simulink model "c00006M_harness"  (R2018a)
settings: Solver=FixedStepAuto  StartTime=0.0  StopTime=300  FixedStep=0.1  RelTol=1e-3
undefined symbols (not defined in the file): A1, hmax, PriorityTank, R1, R2, sigbuilder_block, TempThreshold
(part 1 of 66)
settings Model: Creator=aarrieta  LastModifiedBy=umarkiegi

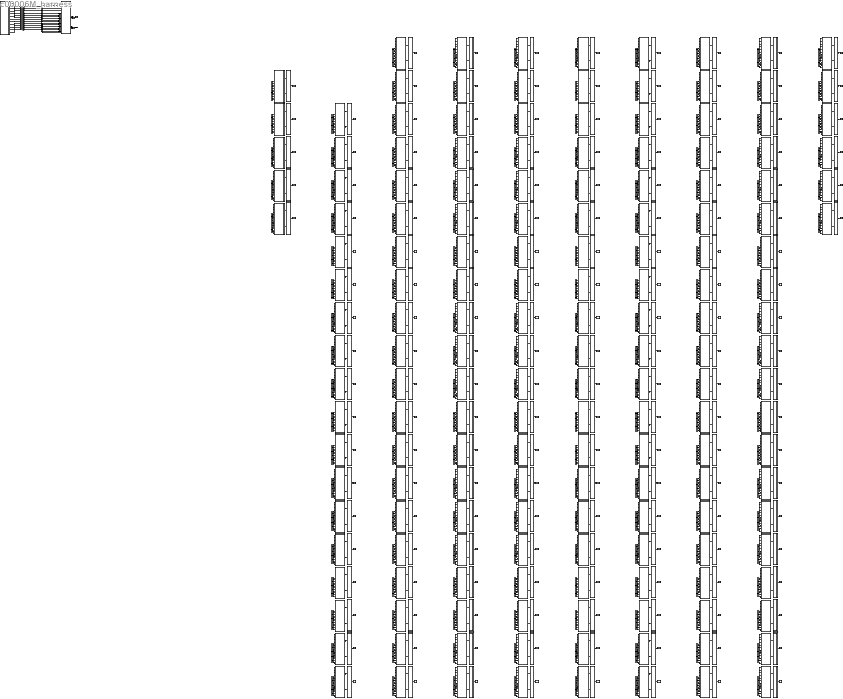
== system c00006M_harness ==
  CPSUT : Subsystem
  Eval100 : Subsystem
  Eval101 : Subsystem
  Eval102 : Subsystem
  Eval103 : Subsystem
  Eval104 : Subsystem
  Eval105 : Subsystem
  Eval106 : Subsystem
  Eval107 : Subsystem
  Eval108 : Subsystem
  Eval109 : Subsystem
  Eval110 : Subsystem
  Eval111 : Subsystem
  Eval112 : Subsystem
  Eval113 : Subsystem
  Eval114 : Subsystem
  Eval115 : Subsystem
  Eval116 : Subsystem
  Eval117 : Subsystem
  Eval118 : Subsystem
  Eval119 : Subsystem
  Eval120 : Subsystem
  Eval121 : Subsystem
  Eval122 : Subsystem
  Eval123 : Subsystem
  Eval124 : Subsystem
  Eval125 : Subsystem
  Eval126 : Subsystem
  Eval127 : Subsystem
  Eval128 : Subsystem
  Eval129 : Subsystem
  Eval130 : Subsystem
  Eval131 : Subsystem
  Eval132 : Subsystem
  Eval133 : Subsystem
  Eval134 : Subsystem
  Eval135 : Subsystem
  Eval136 : Subsystem
  Eval137 : Subsystem
  Eval138 : Subsystem
  Eval139 : Subsystem
  Eval140 : Subsystem
  Eval141 : Subsystem
  Eval142 : Subsystem
  Eval143 : Subsystem
  Eval144 : Subsystem
  Eval145 : Subsystem
  Eval146 : Subsystem
  Eval147 : Subsystem
  Eval148 : Subsystem
  Eval149 : Subsystem
  Eval150 : Subsystem
  Eval151 : Subsystem
  Eval152 : Subsystem
  Eval153 : Subsystem
  Eval154 : Subsystem
  Eval155 : Subsystem
  Eval156 : Subsystem
  Eval157 : Subsystem
  Eval158 : Subsystem
  Eval159 : Subsystem
  Eval160 : Subsystem
  Eval161 : Subsystem
  Eval162 : Subsystem
  Eval163 : Subsystem
  Eval164 : Subsystem
  Eval165 : Subsystem
  Eval166 : Subsystem
  Eval167 : Subsystem
  Eval168 : Subsystem
  Eval169 : Subsystem
  Eval170 : Subsystem
  Eval171 : Subsystem
  Eval172 : Subsystem
  Eval173 : Subsystem
  Eval174 : Subsystem
  Eval175 : Subsystem
  Eval176 : Subsystem
  Eval177 : Subsystem
  Eval178 : Subsystem
  Eval179 : Subsystem
  Eval180 : Subsystem
  Eval181 : Subsystem
  Eval182 : Subsystem
  Eval183 : Subsystem
  Eval184 : Subsystem
  Eval185 : Subsystem
  Eval186 : Subsystem
  Eval187 : Subsystem
  Eval188 : Subsystem
  Eval189 : Subsystem
  Eval190 : Subsystem
  Eval191 : Subsystem
  Eval192 : Subsystem
  Eval193 : Subsystem
  Eval194 : Subsystem
  Eval195 : Subsystem
  Eval196 : Subsystem
  Eval197 : Subsystem
  Eval198 : Subsystem
  Eval199 : Subsystem
  Eval200 : Subsystem
  Eval201 : Subsystem
  Eval202 : Subsystem
  Eval203 : Subsystem
  Eval204 : Subsystem
  Eval205 : Subsystem
  Eval206 : Subsystem
  Eval207 : Subsystem
  Eval208 : Subsystem
  Eval209 : Subsystem
  Eval210 : Subsystem
  Eval211 : Subsystem
  Eval212 : Subsystem
  Eval213 : Subsystem
  Eval214 : Subsystem
  Eval215 : Subsystem
  Eval216 : Subsystem
  Eval217 : Subsystem
  Eval218 : Subsystem
  Eval219 : Subsystem
  Eval220 : Subsystem
  Eval221 : Subsystem
  Eval222 : Subsystem
  Eval223 : Subsystem
  Eval224 : Subsystem
  Eval225 : Subsystem
  Eval226 : Subsystem
  Eval227 : Subsystem
  Eval228 : Subsystem
  Eval229 : Subsystem
  Eval230 : Subsystem
  Eval231 : Subsystem
  Eval232 : Subsystem
  Eval233 : Subsystem
  Eval234 : Subsystem
  Eval235 : Subsystem
  Eval236 : Subsystem
  Eval237 : Subsystem
  Eval238 : Subsystem
  Eval239 : Subsystem
  Eval240 : Subsystem
  Eval241 : Subsystem
  Eval242 : Subsystem
  Eval243 : Subsystem
  Eval244 : Subsystem
  Eval245 : Subsystem
  Eval61 : Subsystem
  Eval62 : Subsystem
  Eval63 : Subsystem
  Eval64 : Subsystem
  Eval65 : Subsystem
  Eval82 : Subsystem
  Eval83 : Subsystem
  Eval84 : Subsystem
  Eval85 : Subsystem
  Eval86 : Subsystem
  Eval87 : Subsystem
  Eval88 : Subsystem
  Eval89 : Subsystem
  Eval90 : Subsystem
  Eval91 : Subsystem
  Eval92 : Subsystem
  Eval93 : Subsystem
  Eval94 : Subsystem
  Eval95 : Subsystem
  Eval96 : Subsystem
  Eval97 : Subsystem
  Eval98 : Subsystem
  Eval99 : Subsystem
  Inputs : Subsystem  Tag=STV Subsys  LoadFcn=sigbuilder_block('load');  StartFcn=sigbuilder_block('start');  StopFcn=sigbuilder_block('stop');  ClipboardFcn=sigbuilder_block('clipboard');  mask(Sigbuilder block){tuvar=[0:10]}
      mask init:
      | if ~strcmp(get_param(bdroot(gcb),'SimulationStatus'),'stopped'),tuvar = sigbuilder_block('maskInit'); end
      settings: CopyFcn=sigbuilder_block('copy');  DeleteFcn=sigbuilder_block('delete');  ModelCloseFcn=sigbuilder_block('modelClose');  PreSaveFcn=sigbuilder_block('preSave');  PauseFcn=sigbuilder_block('pause');  ContinueFcn=sigbuilder_block('continue');  NameChangeFcn=sigbuilder_block('namechange');  OpenFcn=sigbuilder_block('open',[276.75 163.5 675.75 486.75 ]);  CloseFcn=sigbuilder_block('close');
      mask Display: plot(0, 0, 100, 100,[2, 2, 32, 32, 2], [68, 8, 8, 68, 68],[32, 2], [38, 38], [32, 19, 2],[53, 60, 44], [32, 17, 17, 2],[16, 16, 31, 31]);txt = getActiveGroup(gcbh);text(2, 100, txt,'verticalAlignment', 'top');
  M062 : Subsystem
  M063 : Subsystem
  M064 : Subsystem
  M065 : Subsystem
  M066 : Subsystem
  M083 : Subsystem
  M084 : Subsystem
  M085 : Subsystem
  M086 : Subsystem
  M087 : Subsystem
  M088 : Subsystem
  M089 : Subsystem
  M090 : Subsystem
  M091 : Subsystem
  M092 : Subsystem
  M093 : Subsystem
  M094 : Subsystem
  M095 : Subsystem
  M096 : Subsystem
  M097 : Subsystem
  M098 : Subsystem
  M099 : Subsystem
  M100 : Subsystem
  M101 : Subsystem
  M102 : Subsystem
  M103 : Subsystem
  M104 : Subsystem
  M105 : Subsystem
  M106 : Subsystem
  M107 : Subsystem
  M108 : Subsystem
  M109 : Subsystem
  M110 : Subsystem
  M111 : Subsystem
  M112 : Subsystem
  M113 : Subsystem
  M114 : Subsystem
  M115 : Subsystem
  M116 : Subsystem
  M117 : Subsystem
  M118 : Subsystem
  M119 : Subsystem
  M120 : Subsystem
  M121 : Subsystem
  M122 : Subsystem
  M123 : Subsystem
  M124 : Subsystem
  M125 : Subsystem
  M126 : Subsystem
  M127 : Subsystem
  M128 : Subsystem
  M129 : Subsystem
  M130 : Subsystem
  M131 : Subsystem
  M132 : Subsystem
  M133 : Subsystem
  M134 : Subsystem
  M135 : Subsystem
  M136 : Subsystem
  M137 : Subsystem
  M138 : Subsystem
  M139 : Subsystem
  M140 : Subsystem
  M141 : Subsystem
  M142 : Subsystem
  M143 : Subsystem
  M144 : Subsystem
  M145 : Subsystem
  M146 : Subsystem
  M147 : Subsystem
  M148 : Subsystem
  M149 : Subsystem
  M150 : Subsystem
  M151 : Subsystem
  M152 : Subsystem
  M153 : Subsystem
  M154 : Subsystem
  M155 : Subsystem
  M156 : Subsystem
  M157 : Subsystem
  M158 : Subsystem
  M159 : Subsystem
  M160 : Subsystem
  M161 : Subsystem
  M162 : Subsystem
  M163 : Subsystem
  M164 : Subsystem
  M165 : Subsystem
  M166 : Subsystem
  M167 : Subsystem
  M168 : Subsystem
  M169 : Subsystem
  M170 : Subsystem
  M171 : Subsystem
  M172 : Subsystem
  M173 : Subsystem
  M174 : Subsystem
  M175 : Subsystem
  M176 : Subsystem
  M177 : Subsystem
  M178 : Subsystem
  M179 : Subsystem
  M180 : Subsystem
  M181 : Subsystem
  M182 : Subsystem
  M183 : Subsystem
  M184 : Subsystem
  M185 : Subsystem
  M186 : Subsystem
  M187 : Subsystem
  M188 : Subsystem
  M189 : Subsystem
  M190 : Subsystem
  M191 : Subsystem
  M192 : Subsystem
  M193 : Subsystem
  M194 : Subsystem
  M195 : Subsystem
  M196 : Subsystem
  M197 : Subsystem
  M198 : Subsystem
  M199 : Subsystem
  M200 : Subsystem
  M201 : Subsystem
  M202 : Subsystem
  M203 : Subsystem
  M204 : Subsystem
  M205 : Subsystem
  M206 : Subsystem
  M207 : Subsystem
  M208 : Subsystem
  M209 : Subsystem
  M210 : Subsystem
  M211 : Subsystem
  M212 : Subsystem
  M213 : Subsystem
  M214 : Subsystem
  M215 : Subsystem
  M216 : Subsystem
  M217 : Subsystem
  M218 : Subsystem
  M219 : Subsystem
  M220 : Subsystem
  M221 : Subsystem
  M222 : Subsystem
  M223 : Subsystem
  M224 : Subsystem
  M225 : Subsystem
  M226 : Subsystem
  M227 : Subsystem
  M228 : Subsystem
  M229 : Subsystem
  M230 : Subsystem
  M231 : Subsystem
  M232 : Subsystem
  M233 : Subsystem
  M234 : Subsystem
  M235 : Subsystem
  M236 : Subsystem
  M237 : Subsystem
  M238 : Subsystem
  M239 : Subsystem
  M240 : Subsystem
  M241 : Subsystem
  M242 : Subsystem
  M243 : Subsystem
  M244 : Subsystem
  M245 : Subsystem
  M246 : Subsystem
  To Workspace100 : ToWorkspace  VariableName=mutant101  SampleTime=-1
  To Workspace101 : ToWorkspace  VariableName=mutant102  SampleTime=-1
  To Workspace102 : ToWorkspace  VariableName=mutant103  SampleTime=-1
  To Workspace103 : ToWorkspace  VariableName=mutant104  SampleTime=-1
  To Workspace104 : ToWorkspace  VariableName=mutant105  SampleTime=-1
  To Workspace105 : ToWorkspace  VariableName=mutant106  SampleTime=-1
  To Workspace106 : ToWorkspace  VariableName=mutant107  SampleTime=-1
  To Workspace107 : ToWorkspace  VariableName=mutant108  SampleTime=-1
  To Workspace108 : ToWorkspace  VariableName=mutant109  SampleTime=-1
  To Workspace109 : ToWorkspace  VariableName=mutant110  SampleTime=-1
  To Workspace110 : ToWorkspace  VariableName=mutant111  SampleTime=-1
  To Workspace111 : ToWorkspace  VariableName=mutant112  SampleTime=-1
  To Workspace112 : ToWorkspace  VariableName=mutant113  SampleTime=-1
  To Workspace113 : ToWorkspace  VariableName=mutant114  SampleTime=-1
  To Workspace114 : ToWorkspace  VariableName=mutant115  SampleTime=-1
  To Workspace115 : ToWorkspace  VariableName=mutant116  SampleTime=-1
  To Workspace116 : ToWorkspace  VariableName=mutant117  SampleTime=-1
  To Workspace117 : ToWorkspace  VariableName=mutant118  SampleTime=-1
  To Workspace118 : ToWorkspace  VariableName=mutant119  SampleTime=-1
  To Workspace119 : ToWorkspace  VariableName=mutant120  SampleTime=-1
  To Workspace120 : ToWorkspace  VariableName=mutant121  SampleTime=-1
  To Workspace121 : ToWorkspace  VariableName=mutant122  SampleTime=-1
  To Workspace122 : ToWorkspace  VariableName=mutant123  SampleTime=-1
  To Workspace123 : ToWorkspace  VariableName=mutant124  SampleTime=-1
  To Workspace124 : ToWorkspace  VariableName=mutant125  SampleTime=-1
  To Workspace125 : ToWorkspace  VariableName=mutant126  SampleTime=-1
  To Workspace126 : ToWorkspace  VariableName=mutant127  SampleTime=-1
  To Workspace127 : ToWorkspace  VariableName=mutant128  SampleTime=-1
  To Workspace128 : ToWorkspace  VariableName=mutant129  SampleTime=-1
  To Workspace129 : ToWorkspace  VariableName=mutant130  SampleTime=-1
  To Workspace130 : ToWorkspace  VariableName=mutant131  SampleTime=-1
  To Workspace131 : ToWorkspace  VariableName=mutant132  SampleTime=-1
  To Workspace132 : ToWorkspace  VariableName=mutant133  SampleTime=-1
  To Workspace133 : ToWorkspace  VariableName=mutant134  SampleTime=-1
  To Workspace134 : ToWorkspace  VariableName=mutant135  SampleTime=-1
  To Workspace135 : ToWorkspace  VariableName=mutant136  SampleTime=-1
  To Workspace136 : ToWorkspace  VariableName=mutant137  SampleTime=-1
  To Workspace137 : ToWorkspace  VariableName=mutant138  SampleTime=-1
  To Workspace138 : ToWorkspace  VariableName=mutant139  SampleTime=-1
  To Workspace139 : ToWorkspace  VariableName=mutant140  SampleTime=-1
  To Workspace140 : ToWorkspace  VariableName=mutant141  SampleTime=-1
  To Workspace141 : ToWorkspace  VariableName=mutant142  SampleTime=-1
  To Workspace142 : ToWorkspace  VariableName=mutant143  SampleTime=-1
  To Workspace143 : ToWorkspace  VariableName=mutant144  SampleTime=-1
  To Workspace144 : ToWorkspace  VariableName=mutant145  SampleTime=-1
  To Workspace145 : ToWorkspace  VariableName=mutant146  SampleTime=-1
  To Workspace146 : ToWorkspace  VariableName=mutant147  SampleTime=-1
  To Workspace147 : ToWorkspace  VariableName=mutant148  SampleTime=-1
  To Workspace148 : ToWorkspace  VariableName=mutant149  SampleTime=-1
  To Workspace149 : ToWorkspace  VariableName=mutant150  SampleTime=-1
  To Workspace150 : ToWorkspace  VariableName=mutant151  SampleTime=-1
  To Workspace151 : ToWorkspace  VariableName=mutant152  SampleTime=-1
  To Workspace152 : ToWorkspace  VariableName=mutant153  SampleTime=-1
  To Workspace153 : ToWorkspace  VariableName=mutant154  SampleTime=-1
  To Workspace154 : ToWorkspace  VariableName=mutant155  SampleTime=-1
  To Workspace155 : ToWorkspace  VariableName=mutant156  SampleTime=-1
  To Workspace156 : ToWorkspace  VariableName=mutant157  SampleTime=-1
  To Workspace157 : ToWorkspace  VariableName=mutant158  SampleTime=-1
  To Workspace158 : ToWorkspace  VariableName=mutant159  SampleTime=-1
  To Workspace159 : ToWorkspace  VariableName=mutant160  SampleTime=-1
  To Workspace160 : ToWorkspace  VariableName=mutant161  SampleTime=-1
  To Workspace161 : ToWorkspace  VariableName=mutant162  SampleTime=-1
  To Workspace162 : ToWorkspace  VariableName=mutant163  SampleTime=-1
  To Workspace163 : ToWorkspace  VariableName=mutant164  SampleTime=-1
  To Workspace164 : ToWorkspace  VariableName=mutant165  SampleTime=-1
  To Workspace165 : ToWorkspace  VariableName=mutant166  SampleTime=-1
  To Workspace166 : ToWorkspace  VariableName=mutant167  SampleTime=-1
  To Workspace167 : ToWorkspace  VariableName=mutant168  SampleTime=-1
  To Workspace168 : ToWorkspace  VariableName=mutant169  SampleTime=-1
  To Workspace169 : ToWorkspace  VariableName=mutant170  SampleTime=-1
  To Workspace170 : ToWorkspace  VariableName=mutant171  SampleTime=-1
  To Workspace171 : ToWorkspace  VariableName=mutant172  SampleTime=-1
  To Workspace172 : ToWorkspace  VariableName=mutant173  SampleTime=-1
  To Workspace173 : ToWorkspace  VariableName=mutant174  SampleTime=-1
  To Workspace174 : ToWorkspace  VariableName=mutant175  SampleTime=-1
  To Workspace175 : ToWorkspace  VariableName=mutant176  SampleTime=-1
  To Workspace176 : ToWorkspace  VariableName=mutant177  SampleTime=-1
  To Workspace177 : ToWorkspace  VariableName=mutant178  SampleTime=-1
  To Workspace178 : ToWorkspace  VariableName=mutant179  SampleTime=-1
  To Workspace179 : ToWorkspace  VariableName=mutant180  SampleTime=-1
  To Workspace180 : ToWorkspace  VariableName=mutant181  SampleTime=-1
  To Workspace181 : ToWorkspace  VariableName=mutant182  SampleTime=-1
  To Workspace182 : ToWorkspace  VariableName=mutant183  SampleTime=-1
  To Workspace183 : ToWorkspace  VariableName=mutant184  SampleTime=-1
  To Workspace184 : ToWorkspace  VariableName=mutant185  SampleTime=-1
  To Workspace185 : ToWorkspace  VariableName=mutant186  SampleTime=-1
  To Workspace186 : ToWorkspace  VariableName=mutant187  SampleTime=-1
  To Workspace187 : ToWorkspace  VariableName=mutant188  SampleTime=-1
  To Workspace188 : ToWorkspace  VariableName=mutant189  SampleTime=-1
  To Workspace189 : ToWorkspace  VariableName=mutant190  SampleTime=-1
  To Workspace190 : ToWorkspace  VariableName=mutant191  SampleTime=-1
  To Workspace191 : ToWorkspace  VariableName=mutant192  SampleTime=-1
  To Workspace192 : ToWorkspace  VariableName=mutant193  SampleTime=-1
  To Workspace193 : ToWorkspace  VariableName=mutant194  SampleTime=-1
  To Workspace194 : ToWorkspace  VariableName=mutant195  SampleTime=-1
  To Workspace195 : ToWorkspace  VariableName=mutant196  SampleTime=-1
  To Workspace196 : ToWorkspace  VariableName=mutant197  SampleTime=-1
  To Workspace197 : ToWorkspace  VariableName=mutant198  SampleTime=-1
  To Workspace198 : ToWorkspace  VariableName=mutant199  SampleTime=-1
  To Workspace199 : ToWorkspace  VariableName=mutant200  SampleTime=-1
  To Workspace200 : ToWorkspace  VariableName=mutant201  SampleTime=-1
  To Workspace201 : ToWorkspace  VariableName=mutant202  SampleTime=-1
  To Workspace202 : ToWorkspace  VariableName=mutant203  SampleTime=-1
  To Workspace203 : ToWorkspace  VariableName=mutant204  SampleTime=-1
  To Workspace204 : ToWorkspace  VariableName=mutant205  SampleTime=-1
  To Workspace205 : ToWorkspace  VariableName=mutant206  SampleTime=-1
  To Workspace206 : ToWorkspace  VariableName=mutant207  SampleTime=-1
  To Workspace207 : ToWorkspace  VariableName=mutant208  SampleTime=-1
  To Workspace208 : ToWorkspace  VariableName=mutant209  SampleTime=-1
  To Workspace209 : ToWorkspace  VariableName=mutant210  SampleTime=-1
  To Workspace210 : ToWorkspace  VariableName=mutant211  SampleTime=-1
  To Workspace211 : ToWorkspace  VariableName=mutant212  SampleTime=-1
  To Workspace212 : ToWorkspace  VariableName=mutant213  SampleTime=-1
  To Workspace213 : ToWorkspace  VariableName=mutant214  SampleTime=-1
  To Workspace214 : ToWorkspace  VariableName=mutant215  SampleTime=-1
  To Workspace215 : ToWorkspace  VariableName=mutant216  SampleTime=-1
  To Workspace216 : ToWorkspace  VariableName=mutant217  SampleTime=-1
  To Workspace217 : ToWorkspace  VariableName=mutant218  SampleTime=-1
  To Workspace218 : ToWorkspace  VariableName=mutant219  SampleTime=-1
  To Workspace219 : ToWorkspace  VariableName=mutant220  SampleTime=-1
  To Workspace220 : ToWorkspace  VariableName=mutant221  SampleTime=-1
  To Workspace221 : ToWorkspace  VariableName=mutant222  SampleTime=-1
  To Workspace222 : ToWorkspace  VariableName=mutant223  SampleTime=-1
  To Workspace223 : ToWorkspace  VariableName=mutant224  SampleTime=-1
  To Workspace224 : ToWorkspace  VariableName=mutant225  SampleTime=-1
  To Workspace225 : ToWorkspace  VariableName=mutant226  SampleTime=-1
  To Workspace226 : ToWorkspace  VariableName=mutant227  SampleTime=-1
  To Workspace227 : ToWorkspace  VariableName=mutant228  SampleTime=-1
  To Workspace228 : ToWorkspace  VariableName=mutant229  SampleTime=-1
  To Workspace229 : ToWorkspace  VariableName=mutant230  SampleTime=-1
  To Workspace230 : ToWorkspace  VariableName=mutant231  SampleTime=-1
  To Workspace231 : ToWorkspace  VariableName=mutant232  SampleTime=-1
  To Workspace232 : ToWorkspace  VariableName=mutant233  SampleTime=-1
  To Workspace233 : ToWorkspace  VariableName=mutant234  SampleTime=-1
  To Workspace234 : ToWorkspace  VariableName=mutant235  SampleTime=-1
  To Workspace235 : ToWorkspace  VariableName=mutant236  SampleTime=-1
  To Workspace236 : ToWorkspace  VariableName=mutant237  SampleTime=-1
  To Workspace237 : ToWorkspace  VariableName=mutant238  SampleTime=-1
  To Workspace238 : ToWorkspace  VariableName=mutant239  SampleTime=-1
  To Workspace239 : ToWorkspace  VariableName=mutant240  SampleTime=-1
  To Workspace240 : ToWorkspace  VariableName=mutant241  SampleTime=-1
  To Workspace241 : ToWorkspace  VariableName=mutant242  SampleTime=-1
  To Workspace242 : ToWorkspace  VariableName=mutant243  SampleTime=-1
  To Workspace243 : ToWorkspace  VariableName=mutant244  SampleTime=-1
  To Workspace244 : ToWorkspace  VariableName=mutant245  SampleTime=-1
  To Workspace245 : ToWorkspace  VariableName=mutant246  SampleTime=-1
  To Workspace61 : ToWorkspace  VariableName=mutant062  SampleTime=-1
  To Workspace62 : ToWorkspace  VariableName=mutant063  SampleTime=-1
  To Workspace63 : ToWorkspace  VariableName=mutant064  SampleTime=-1
  To Workspace64 : ToWorkspace  VariableName=mutant065  SampleTime=-1
  To Workspace65 : ToWorkspace  VariableName=mutant066  SampleTime=-1
  To Workspace82 : ToWorkspace  VariableName=mutant083  SampleTime=-1
  To Workspace83 : ToWorkspace  VariableName=mutant084  SampleTime=-1
  To Workspace84 : ToWorkspace  VariableName=mutant085  SampleTime=-1
  To Workspace85 : ToWorkspace  VariableName=mutant086  SampleTime=-1
  To Workspace86 : ToWorkspace  VariableName=mutant087  SampleTime=-1
  To Workspace87 : ToWorkspace  VariableName=mutant088  SampleTime=-1
  To Workspace88 : ToWorkspace  VariableName=mutant089  SampleTime=-1
  To Workspace89 : ToWorkspace  VariableName=mutant090  SampleTime=-1
  To Workspace90 : ToWorkspace  VariableName=mutant091  SampleTime=-1
  To Workspace91 : ToWorkspace  VariableName=mutant092  SampleTime=-1
  To Workspace92 : ToWorkspace  VariableName=mutant093  SampleTime=-1
  To Workspace93 : ToWorkspace  VariableName=mutant094  SampleTime=-1
  To Workspace94 : ToWorkspace  VariableName=mutant095  SampleTime=-1
  To Workspace95 : ToWorkspace  VariableName=mutant096  SampleTime=-1
  To Workspace96 : ToWorkspace  VariableName=mutant097  SampleTime=-1
  To Workspace97 : ToWorkspace  VariableName=mutant098  SampleTime=-1
  To Workspace98 : ToWorkspace  VariableName=mutant099  SampleTime=-1
  To Workspace99 : ToWorkspace  VariableName=mutant100  SampleTime=-1
  dtc_CT2 : DataTypeConversion
  dtc_CT3 : DataTypeConversion
  dtc_E2 : DataTypeConversion
  dtc_E3 : DataTypeConversion
  dtc_EB2 : DataTypeConversion
  dtc_EB3 : DataTypeConversion
  dtc_F2 : DataTypeConversion
  dtc_F3 : DataTypeConversion
  dtc_MR2 : DataTypeConversion
  dtc_MR3 : DataTypeConversion
  dtc_T2 : DataTypeConversion
  dtc_T3 : DataTypeConversion
  LL2 : Outport
  LL3 : Outport  Port=2
  tag scope: out2=global, out3=global
  wires:
  CPSUT/1(LL2) -> [out2], LL2/1
  CPSUT/2(LL3) -> [out3], LL3/1
  [in7] -> M062/1(CT2)
  [in8] -> M062/2(F2)
  [in9] -> M062/3(E2)
  [in10] -> M062/4(MR2)
  [in11] -> M062/5(T2)
  [in12] -> M062/6(EB2)
  [in13] -> M062/7(CT3)
  [in14] -> M062/8(F3)
  [in15] -> M062/9(E3)
  [in16] -> M062/10(MR3)
  [in17] -> M062/11(T3)
  [in18] -> M062/12(EB3)
  M062/1(LL2) -> Eval61/1(In2)
  M062/2(LL3) -> Eval61/2(In3)
  Eval61/1(Out1) -> To Workspace61/1
  [in7] -> M063/1(CT2)
  [in8] -> M063/2(F2)
  [in9] -> M063/3(E2)
  [in10] -> M063/4(MR2)
  [in11] -> M063/5(T2)
  [in12] -> M063/6(EB2)
  [in13] -> M063/7(CT3)
  [in14] -> M063/8(F3)
  [in15] -> M063/9(E3)
  [in16] -> M063/10(MR3)
  [in17] -> M063/11(T3)
  [in18] -> M063/12(EB3)
  M063/1(LL2) -> Eval62/1(In2)
  M063/2(LL3) -> Eval62/2(In3)
  Eval62/1(Out1) -> To Workspace62/1
  [in7] -> M064/1(CT2)
  [in8] -> M064/2(F2)
  [in9] -> M064/3(E2)
  [in10] -> M064/4(MR2)
  [in11] -> M064/5(T2)
  [in12] -> M064/6(EB2)
  [in13] -> M064/7(CT3)
  [in14] -> M064/8(F3)
  [in15] -> M064/9(E3)
  [in16] -> M064/10(MR3)
  [in17] -> M064/11(T3)
  [in18] -> M064/12(EB3)
  M064/1(LL2) -> Eval63/1(In2)
  M064/2(LL3) -> Eval63/2(In3)
  Eval63/1(Out1) -> To Workspace63/1
  [in7] -> M065/1(CT2)
  [in8] -> M065/2(F2)
  [in9] -> M065/3(E2)
  [in10] -> M065/4(MR2)
  [in11] -> M065/5(T2)
  [in12] -> M065/6(EB2)
  [in13] -> M065/7(CT3)
  [in14] -> M065/8(F3)
  [in15] -> M065/9(E3)
  [in16] -> M065/10(MR3)
  [in17] -> M065/11(T3)
  [in18] -> M065/12(EB3)
  M065/1(LL2) -> Eval64/1(In2)
  M065/2(LL3) -> Eval64/2(In3)
  Eval64/1(Out1) -> To Workspace64/1
  [in7] -> M066/1(CT2)
  [in8] -> M066/2(F2)
  [in9] -> M066/3(E2)
  [in10] -> M066/4(MR2)
  [in11] -> M066/5(T2)
  [in12] -> M066/6(EB2)
  [in13] -> M066/7(CT3)
  [in14] -> M066/8(F3)
  [in15] -> M066/9(E3)
  [in16] -> M066/10(MR3)
  [in17] -> M066/11(T3)
  [in18] -> M066/12(EB3)
  M066/1(LL2) -> Eval65/1(In2)
  M066/2(LL3) -> Eval65/2(In3)
  Eval65/1(Out1) -> To Workspace65/1
  [in7] -> M083/1(CT2)
  [in8] -> M083/2(F2)
  [in9] -> M083/3(E2)
  [in10] -> M083/4(MR2)
  [in11] -> M083/5(T2)
  [in12] -> M083/6(EB2)
  [in13] -> M083/7(CT3)
  [in14] -> M083/8(F3)
  [in15] -> M083/9(E3)
  [in16] -> M083/10(MR3)
  [in17] -> M083/11(T3)
  [in18] -> M083/12(EB3)
  M083/1(LL2) -> Eval82/1(In2)
  M083/2(LL3) -> Eval82/2(In3)
  Eval82/1(Out1) -> To Workspace82/1
  [in7] -> M084/1(CT2)
  [in8] -> M084/2(F2)
  [in9] -> M084/3(E2)
  [in10] -> M084/4(MR2)
  [in11] -> M084/5(T2)
  [in12] -> M084/6(EB2)
  [in13] -> M084/7(CT3)
  [in14] -> M084/8(F3)
  [in15] -> M084/9(E3)
  [in16] -> M084/10(MR3)
  [in17] -> M084/11(T3)
  [in18] -> M084/12(EB3)
  M084/1(LL2) -> Eval83/1(In2)
  M084/2(LL3) -> Eval83/2(In3)
  Eval83/1(Out1) -> To Workspace83/1
  [in7] -> M085/1(CT2)
  [in8] -> M085/2(F2)
  [in9] -> M085/3(E2)
  [in10] -> M085/4(MR2)
  [in11] -> M085/5(T2)
  [in12] -> M085/6(EB2)
  [in13] -> M085/7(CT3)
  [in14] -> M085/8(F3)
  [in15] -> M085/9(E3)
  [in16] -> M085/10(MR3)
  [in17] -> M085/11(T3)
  [in18] -> M085/12(EB3)
  M085/1(LL2) -> Eval84/1(In2)
  M085/2(LL3) -> Eval84/2(In3)
  Eval84/1(Out1) -> To Workspace84/1
  [in7] -> M086/1(CT2)
  [in8] -> M086/2(F2)
  [in9] -> M086/3(E2)
  [in10] -> M086/4(MR2)
  [in11] -> M086/5(T2)
  [in12] -> M086/6(EB2)
  [in13] -> M086/7(CT3)
  [in14] -> M086/8(F3)
  [in15] -> M086/9(E3)
  [in16] -> M086/10(MR3)
  [in17] -> M086/11(T3)
  [in18] -> M086/12(EB3)
  M086/1(LL2) -> Eval85/1(In2)
  M086/2(LL3) -> Eval85/2(In3)
  Eval85/1(Out1) -> To Workspace85/1
  [in7] -> M087/1(CT2)
  [in8] -> M087/2(F2)
  [in9] -> M087/3(E2)
  [in10] -> M087/4(MR2)
  [in11] -> M087/5(T2)
  [in12] -> M087/6(EB2)
  [in13] -> M087/7(CT3)
  [in14] -> M087/8(F3)
  [in15] -> M087/9(E3)
  [in16] -> M087/10(MR3)
  [in17] -> M087/11(T3)
  [in18] -> M087/12(EB3)
  M087/1(LL2) -> Eval86/1(In2)
  M087/2(LL3) -> Eval86/2(In3)
  Eval86/1(Out1) -> To Workspace86/1
  [in7] -> M088/1(CT2)
  [in8] -> M088/2(F2)
  [in9] -> M088/3(E2)
  [in10] -> M088/4(MR2)
  [in11] -> M088/5(T2)
  [in12] -> M088/6(EB2)
  [in13] -> M088/7(CT3)
  [in14] -> M088/8(F3)
  [in15] -> M088/9(E3)
  [in16] -> M088/10(MR3)
  [in17] -> M088/11(T3)
  [in18] -> M088/12(EB3)
  M088/1(LL2) -> Eval87/1(In2)
  M088/2(LL3) -> Eval87/2(In3)
  Eval87/1(Out1) -> To Workspace87/1
  [in7] -> M089/1(CT2)
  [in8] -> M089/2(F2)
  [in9] -> M089/3(E2)
  [in10] -> M089/4(MR2)
  [in11] -> M089/5(T2)
  [in12] -> M089/6(EB2)
  [in13] -> M089/7(CT3)
  [in14] -> M089/8(F3)
  [in15] -> M089/9(E3)
  [in16] -> M089/10(MR3)
  [in17] -> M089/11(T3)
  [in18] -> M089/12(EB3)
  M089/1(LL2) -> Eval88/1(In2)
  M089/2(LL3) -> Eval88/2(In3)
  Eval88/1(Out1) -> To Workspace88/1
  [in7] -> M090/1(CT2)
  [in8] -> M090/2(F2)
  [in9] -> M090/3(E2)
  [in10] -> M090/4(MR2)
  [in11] -> M090/5(T2)
  [in12] -> M090/6(EB2)
  [in13] -> M090/7(CT3)
  [in14] -> M090/8(F3)
  [in15] -> M090/9(E3)
  [in16] -> M090/10(MR3)
  [in17] -> M090/11(T3)
  [in18] -> M090/12(EB3)
  M090/1(LL2) -> Eval89/1(In2)
  M090/2(LL3) -> Eval89/2(In3)
  Eval89/1(Out1) -> To Workspace89/1
  [in7] -> M091/1(CT2)
  [in8] -> M091/2(F2)
  [in9] -> M091/3(E2)
  [in10] -> M091/4(MR2)
  [in11] -> M091/5(T2)
  [in12] -> M091/6(EB2)
  [in13] -> M091/7(CT3)
  [in14] -> M091/8(F3)
  [in15] -> M091/9(E3)
  [in16] -> M091/10(MR3)
  [in17] -> M091/11(T3)
  [in18] -> M091/12(EB3)
  M091/1(LL2) -> Eval90/1(In2)
  M091/2(LL3) -> Eval90/2(In3)
  Eval90/1(Out1) -> To Workspace90/1
  [in7] -> M092/1(CT2)
  [in8] -> M092/2(F2)
  [in9] -> M092/3(E2)
  [in10] -> M092/4(MR2)
  [in11] -> M092/5(T2)
  [in12] -> M092/6(EB2)
  [in13] -> M092/7(CT3)
  [in14] -> M092/8(F3)
  [in15] -> M092/9(E3)
  [in16] -> M092/10(MR3)
  [in17] -> M092/11(T3)
  [in18] -> M092/12(EB3)
  M092/1(LL2) -> Eval91/1(In2)
  M092/2(LL3) -> Eval91/2(In3)
  Eval91/1(Out1) -> To Workspace91/1
  [in7] -> M093/1(CT2)
  [in8] -> M093/2(F2)
  [in9] -> M093/3(E2)
  [in10] -> M093/4(MR2)
  [in11] -> M093/5(T2)
  [in12] -> M093/6(EB2)
  [in13] -> M093/7(CT3)
  [in14] -> M093/8(F3)
  [in15] -> M093/9(E3)
  [in16] -> M093/10(MR3)
  [in17] -> M093/11(T3)
  [in18] -> M093/12(EB3)
  M093/1(LL2) -> Eval92/1(In2)
  M093/2(LL3) -> Eval92/2(In3)
  Eval92/1(Out1) -> To Workspace92/1
  [in7] -> M094/1(CT2)
  [in8] -> M094/2(F2)
  [in9] -> M094/3(E2)
  [in10] -> M094/4(MR2)
  [in11] -> M094/5(T2)
  [in12] -> M094/6(EB2)
  [in13] -> M094/7(CT3)
  [in14] -> M094/8(F3)
  [in15] -> M094/9(E3)
  [in16] -> M094/10(MR3)
  [in17] -> M094/11(T3)
  [in18] -> M094/12(EB3)
  M094/1(LL2) -> Eval93/1(In2)
  M094/2(LL3) -> Eval93/2(In3)
  Eval93/1(Out1) -> To Workspace93/1
  [in7] -> M095/1(CT2)
  [in8] -> M095/2(F2)
  [in9] -> M095/3(E2)
  [in10] -> M095/4(MR2)
  [in11] -> M095/5(T2)
  [in12] -> M095/6(EB2)
  [in13] -> M095/7(CT3)
  [in14] -> M095/8(F3)
  [in15] -> M095/9(E3)
  [in16] -> M095/10(MR3)
  [in17] -> M095/11(T3)
  [in18] -> M095/12(EB3)
  M095/1(LL2) -> Eval94/1(In2)
  M095/2(LL3) -> Eval94/2(In3)
  Eval94/1(Out1) -> To Workspace94/1
  [in7] -> M096/1(CT2)
  [in8] -> M096/2(F2)
  [in9] -> M096/3(E2)
  [in10] -> M096/4(MR2)
  [in11] -> M096/5(T2)
  [in12] -> M096/6(EB2)
  [in13] -> M096/7(CT3)
  [in14] -> M096/8(F3)
  [in15] -> M096/9(E3)
  [in16] -> M096/10(MR3)
  [in17] -> M096/11(T3)
  [in18] -> M096/12(EB3)
  M096/1(LL2) -> Eval95/1(In2)
  M096/2(LL3) -> Eval95/2(In3)
  Eval95/1(Out1) -> To Workspace95/1
  [in7] -> M097/1(CT2)
  [in8] -> M097/2(F2)
  [in9] -> M097/3(E2)
  [in10] -> M097/4(MR2)
  [in11] -> M097/5(T2)
  [in12] -> M097/6(EB2)
  [in13] -> M097/7(CT3)
  [in14] -> M097/8(F3)
  [in15] -> M097/9(E3)
  [in16] -> M097/10(MR3)
  [in17] -> M097/11(T3)
  [in18] -> M097/12(EB3)
  M097/1(LL2) -> Eval96/1(In2)
  M097/2(LL3) -> Eval96/2(In3)
  Eval96/1(Out1) -> To Workspace96/1
  [in7] -> M098/1(CT2)
  [in8] -> M098/2(F2)
  [in9] -> M098/3(E2)
  [in10] -> M098/4(MR2)
  [in11] -> M098/5(T2)
  [in12] -> M098/6(EB2)
  [in13] -> M098/7(CT3)
  [in14] -> M098/8(F3)
  [in15] -> M098/9(E3)
  [in16] -> M098/10(MR3)
  [in17] -> M098/11(T3)
  [in18] -> M098/12(EB3)
  M098/1(LL2) -> Eval97/1(In2)
  M098/2(LL3) -> Eval97/2(In3)
  Eval97/1(Out1) -> To Workspace97/1
  [in7] -> M099/1(CT2)
  [in8] -> M099/2(F2)
  [in9] -> M099/3(E2)
  [in10] -> M099/4(MR2)
  [in11] -> M099/5(T2)
  [in12] -> M099/6(EB2)
  [in13] -> M099/7(CT3)
  [in14] -> M099/8(F3)
  [in15] -> M099/9(E3)
  [in16] -> M099/10(MR3)
  [in17] -> M099/11(T3)
  [in18] -> M099/12(EB3)
  M099/1(LL2) -> Eval98/1(In2)
  M099/2(LL3) -> Eval98/2(In3)
  Eval98/1(Out1) -> To Workspace98/1
  [in7] -> M100/1(CT2)
  [in8] -> M100/2(F2)
  [in9] -> M100/3(E2)
  [in10] -> M100/4(MR2)
  [in11] -> M100/5(T2)
  [in12] -> M100/6(EB2)
  [in13] -> M100/7(CT3)
  [in14] -> M100/8(F3)
  [in15] -> M100/9(E3)
  [in16] -> M100/10(MR3)
  [in17] -> M100/11(T3)
  [in18] -> M100/12(EB3)
  M100/1(LL2) -> Eval99/1(In2)
  M100/2(LL3) -> Eval99/2(In3)
  Eval99/1(Out1) -> To Workspace99/1
  [in7] -> M101/1(CT2)
  [in8] -> M101/2(F2)
  [in9] -> M101/3(E2)
  [in10] -> M101/4(MR2)
  [in11] -> M101/5(T2)
  [in12] -> M101/6(EB2)
  [in13] -> M101/7(CT3)
  [in14] -> M101/8(F3)
  [in15] -> M101/9(E3)
  [in16] -> M101/10(MR3)
  [in17] -> M101/11(T3)
  [in18] -> M101/12(EB3)
  M101/1(LL2) -> Eval100/1(In2)
  M101/2(LL3) -> Eval100/2(In3)
  Eval100/1(Out1) -> To Workspace100/1
  [in7] -> M102/1(CT2)
  [in8] -> M102/2(F2)
  [in9] -> M102/3(E2)
  [in10] -> M102/4(MR2)
  [in11] -> M102/5(T2)
  [in12] -> M102/6(EB2)
  [in13] -> M102/7(CT3)
  [in14] -> M102/8(F3)
  [in15] -> M102/9(E3)
  [in16] -> M102/10(MR3)
  [in17] -> M102/11(T3)
  [in18] -> M102/12(EB3)
  M102/1(LL2) -> Eval101/1(In2)
  M102/2(LL3) -> Eval101/2(In3)
  Eval101/1(Out1) -> To Workspace101/1
  [in7] -> M103/1(CT2)
  [in8] -> M103/2(F2)
  [in9] -> M103/3(E2)
  [in10] -> M103/4(MR2)
  [in11] -> M103/5(T2)
  [in12] -> M103/6(EB2)
  [in13] -> M103/7(CT3)
  [in14] -> M103/8(F3)
  [in15] -> M103/9(E3)
  [in16] -> M103/10(MR3)
  [in17] -> M103/11(T3)
  [in18] -> M103/12(EB3)
  M103/1(LL2) -> Eval102/1(In2)
  M103/2(LL3) -> Eval102/2(In3)
  Eval102/1(Out1) -> To Workspace102/1
  [in7] -> M104/1(CT2)
  [in8] -> M104/2(F2)
  [in9] -> M104/3(E2)
  [in10] -> M104/4(MR2)
  [in11] -> M104/5(T2)
  [in12] -> M104/6(EB2)
  [in13] -> M104/7(CT3)
  [in14] -> M104/8(F3)
  [in15] -> M104/9(E3)
  [in16] -> M104/10(MR3)
  [in17] -> M104/11(T3)
  [in18] -> M104/12(EB3)
  M104/1(LL2) -> Eval103/1(In2)
  M104/2(LL3) -> Eval103/2(In3)
  Eval103/1(Out1) -> To Workspace103/1
  [in7] -> M105/1(CT2)
  [in8] -> M105/2(F2)
  [in9] -> M105/3(E2)
  [in10] -> M105/4(MR2)
  [in11] -> M105/5(T2)
  [in12] -> M105/6(EB2)
  [in13] -> M105/7(CT3)
  [in14] -> M105/8(F3)
  [in15] -> M105/9(E3)
  [in16] -> M105/10(MR3)
  [in17] -> M105/11(T3)
  [in18] -> M105/12(EB3)
  M105/1(LL2) -> Eval104/1(In2)
  M105/2(LL3) -> Eval104/2(In3)
  Eval104/1(Out1) -> To Workspace104/1
  [in7] -> M106/1(CT2)
  [in8] -> M106/2(F2)
  [in9] -> M106/3(E2)
  [in10] -> M106/4(MR2)
  [in11] -> M106/5(T2)
  [in12] -> M106/6(EB2)
  [in13] -> M106/7(CT3)
  [in14] -> M106/8(F3)
  [in15] -> M106/9(E3)
  [in16] -> M106/10(MR3)
  [in17] -> M106/11(T3)
  [in18] -> M106/12(EB3)
  M106/1(LL2) -> Eval105/1(In2)
  M106/2(LL3) -> Eval105/2(In3)
  Eval105/1(Out1) -> To Workspace105/1
  [in7] -> M107/1(CT2)
  [in8] -> M107/2(F2)
  [in9] -> M107/3(E2)
  [in10] -> M107/4(MR2)
  [in11] -> M107/5(T2)
  [in12] -> M107/6(EB2)
  [in13] -> M107/7(CT3)
  [in14] -> M107/8(F3)
  [in15] -> M107/9(E3)
  [in16] -> M107/10(MR3)
  [in17] -> M107/11(T3)
  [in18] -> M107/12(EB3)
  M107/1(LL2) -> Eval106/1(In2)
  M107/2(LL3) -> Eval106/2(In3)
  Eval106/1(Out1) -> To Workspace106/1
  [in7] -> M108/1(CT2)
  [in8] -> M108/2(F2)
  [in9] -> M108/3(E2)
  [in10] -> M108/4(MR2)
  [in11] -> M108/5(T2)
  [in12] -> M108/6(EB2)
  [in13] -> M108/7(CT3)
  [in14] -> M108/8(F3)
  [in15] -> M108/9(E3)
  [in16] -> M108/10(MR3)
  [in17] -> M108/11(T3)
  [in18] -> M108/12(EB3)
  M108/1(LL2) -> Eval107/1(In2)
  M108/2(LL3) -> Eval107/2(In3)
  Eval107/1(Out1) -> To Workspace107/1
  [in7] -> M109/1(CT2)
  [in8] -> M109/2(F2)
  [in9] -> M109/3(E2)
  [in10] -> M109/4(MR2)
  [in11] -> M109/5(T2)
  [in12] -> M109/6(EB2)
  [in13] -> M109/7(CT3)
  [in14] -> M109/8(F3)
  [in15] -> M109/9(E3)
  [in16] -> M109/10(MR3)
  [in17] -> M109/11(T3)
  [in18] -> M109/12(EB3)
  M109/1(LL2) -> Eval108/1(In2)
  M109/2(LL3) -> Eval108/2(In3)
  Eval108/1(Out1) -> To Workspace108/1
  [in7] -> M110/1(CT2)
  [in8] -> M110/2(F2)
  [in9] -> M110/3(E2)
  [in10] -> M110/4(MR2)
  [in11] -> M110/5(T2)
  [in12] -> M110/6(EB2)
  [in13] -> M110/7(CT3)
  [in14] -> M110/8(F3)
  [in15] -> M110/9(E3)
  [in16] -> M110/10(MR3)
  [in17] -> M110/11(T3)
  [in18] -> M110/12(EB3)
  M110/1(LL2) -> Eval109/1(In2)
  M110/2(LL3) -> Eval109/2(In3)
  Eval109/1(Out1) -> To Workspace109/1
  [in7] -> M111/1(CT2)
  [in8] -> M111/2(F2)
  [in9] -> M111/3(E2)
  [in10] -> M111/4(MR2)
  [in11] -> M111/5(T2)
  [in12] -> M111/6(EB2)
  [in13] -> M111/7(CT3)
  [in14] -> M111/8(F3)
  [in15] -> M111/9(E3)
  [in16] -> M111/10(MR3)
  [in17] -> M111/11(T3)
  [in18] -> M111/12(EB3)
  M111/1(LL2) -> Eval110/1(In2)
  M111/2(LL3) -> Eval110/2(In3)
  Eval110/1(Out1) -> To Workspace110/1
  [in7] -> M112/1(CT2)
  [in8] -> M112/2(F2)
  [in9] -> M112/3(E2)
  [in10] -> M112/4(MR2)
  [in11] -> M112/5(T2)
  [in12] -> M112/6(EB2)
  [in13] -> M112/7(CT3)
  [in14] -> M112/8(F3)
  [in15] -> M112/9(E3)
  [in16] -> M112/10(MR3)
  [in17] -> M112/11(T3)
  [in18] -> M112/12(EB3)
  M112/1(LL2) -> Eval111/1(In2)
  M112/2(LL3) -> Eval111/2(In3)
  Eval111/1(Out1) -> To Workspace111/1
  [in7] -> M113/1(CT2)
  [in8] -> M113/2(F2)
  [in9] -> M113/3(E2)
  [in10] -> M113/4(MR2)
  [in11] -> M113/5(T2)
  [in12] -> M113/6(EB2)
  [in13] -> M113/7(CT3)
  [in14] -> M113/8(F3)
  [in15] -> M113/9(E3)
  [in16] -> M113/10(MR3)
  [in17] -> M113/11(T3)
  [in18] -> M113/12(EB3)
  M113/1(LL2) -> Eval112/1(In2)
  M113/2(LL3) -> Eval112/2(In3)
  Eval112/1(Out1) -> To Workspace112/1
  [in7] -> M114/1(CT2)
  [in8] -> M114/2(F2)
  [in9] -> M114/3(E2)
  [in10] -> M114/4(MR2)
  [in11] -> M114/5(T2)
  [in12] -> M114/6(EB2)
  [in13] -> M114/7(CT3)
  [in14] -> M114/8(F3)
  [in15] -> M114/9(E3)
  [in16] -> M114/10(MR3)
  [in17] -> M114/11(T3)
  [in18] -> M114/12(EB3)
  M114/1(LL2) -> Eval113/1(In2)
  M114/2(LL3) -> Eval113/2(In3)
  Eval113/1(Out1) -> To Workspace113/1
  [in7] -> M115/1(CT2)
  [in8] -> M115/2(F2)
  [in9] -> M115/3(E2)
  [in10] -> M115/4(MR2)
  [in11] -> M115/5(T2)
  [in12] -> M115/6(EB2)
  [in13] -> M115/7(CT3)
  [in14] -> M115/8(F3)
  [in15] -> M115/9(E3)
  [in16] -> M115/10(MR3)
  [in17] -> M115/11(T3)
  [in18] -> M115/12(EB3)
  M115/1(LL2) -> Eval114/1(In2)
  M115/2(LL3) -> Eval114/2(In3)
  Eval114/1(Out1) -> To Workspace114/1
  [in7] -> M116/1(CT2)
  [in8] -> M116/2(F2)
  [in9] -> M116/3(E2)
  [in10] -> M116/4(MR2)
  [in11] -> M116/5(T2)
  [in12] -> M116/6(EB2)
  [in13] -> M116/7(CT3)
  [in14] -> M116/8(F3)
  [in15] -> M116/9(E3)
  [in16] -> M116/10(MR3)
  [in17] -> M116/11(T3)
  [in18] -> M116/12(EB3)
  M116/1(LL2) -> Eval115/1(In2)
  M116/2(LL3) -> Eval115/2(In3)
  Eval115/1(Out1) -> To Workspace115/1
  [in7] -> M117/1(CT2)
  [in8] -> M117/2(F2)
  [in9] -> M117/3(E2)
  [in10] -> M117/4(MR2)
  [in11] -> M117/5(T2)
  [in12] -> M117/6(EB2)
  [in13] -> M117/7(CT3)
  [in14] -> M117/8(F3)
  [in15] -> M117/9(E3)
  [in16] -> M117/10(MR3)
  [in17] -> M117/11(T3)
  [in18] -> M117/12(EB3)
  M117/1(LL2) -> Eval116/1(In2)
  M117/2(LL3) -> Eval116/2(In3)
  Eval116/1(Out1) -> To Workspace116/1
  [in7] -> M118/1(CT2)
  [in8] -> M118/2(F2)
  [in9] -> M118/3(E2)
  [in10] -> M118/4(MR2)
  [in11] -> M118/5(T2)
  [in12] -> M118/6(EB2)
  [in13] -> M118/7(CT3)
  [in14] -> M118/8(F3)
  [in15] -> M118/9(E3)
  [in16] -> M118/10(MR3)
  [in17] -> M118/11(T3)
  [in18] -> M118/12(EB3)
  M118/1(LL2) -> Eval117/1(In2)
  M118/2(LL3) -> Eval117/2(In3)
  Eval117/1(Out1) -> To Workspace117/1
  [in7] -> M119/1(CT2)
  [in8] -> M119/2(F2)
  [in9] -> M119/3(E2)
  [in10] -> M119/4(MR2)
  [in11] -> M119/5(T2)
  [in12] -> M119/6(EB2)
  [in13] -> M119/7(CT3)
  [in14] -> M119/8(F3)
  [in15] -> M119/9(E3)
  [in16] -> M119/10(MR3)
  [in17] -> M119/11(T3)
  [in18] -> M119/12(EB3)
  M119/1(LL2) -> Eval118/1(In2)
  M119/2(LL3) -> Eval118/2(In3)
  Eval118/1(Out1) -> To Workspace118/1
  [in7] -> M120/1(CT2)
  [in8] -> M120/2(F2)
  [in9] -> M120/3(E2)
  [in10] -> M120/4(MR2)
  [in11] -> M120/5(T2)
  [in12] -> M120/6(EB2)
  [in13] -> M120/7(CT3)
  [in14] -> M120/8(F3)
  [in15] -> M120/9(E3)
  [in16] -> M120/10(MR3)
  [in17] -> M120/11(T3)
  [in18] -> M120/12(EB3)
  M120/1(LL2) -> Eval119/1(In2)
  M120/2(LL3) -> Eval119/2(In3)
  Eval119/1(Out1) -> To Workspace119/1
  [in7] -> M121/1(CT2)
  [in8] -> M121/2(F2)
  [in9] -> M121/3(E2)
  [in10] -> M121/4(MR2)
  [in11] -> M121/5(T2)
  [in12] -> M121/6(EB2)
  [in13] -> M121/7(CT3)
  [in14] -> M121/8(F3)
  [in15] -> M121/9(E3)
  [in16] -> M121/10(MR3)
  [in17] -> M121/11(T3)
  [in18] -> M121/12(EB3)
  M121/1(LL2) -> Eval120/1(In2)
  M121/2(LL3) -> Eval120/2(In3)
  Eval120/1(Out1) -> To Workspace120/1
  [in7] -> M122/1(CT2)
  [in8] -> M122/2(F2)
  [in9] -> M122/3(E2)
  [in10] -> M122/4(MR2)
  [in11] -> M122/5(T2)
  [in12] -> M122/6(EB2)
  [in13] -> M122/7(CT3)
  [in14] -> M122/8(F3)
  [in15] -> M122/9(E3)
  [in16] -> M122/10(MR3)
  [in17] -> M122/11(T3)
  [in18] -> M122/12(EB3)
  M122/1(LL2) -> Eval121/1(In2)
  M122/2(LL3) -> Eval121/2(In3)
  Eval121/1(Out1) -> To Workspace121/1
  [in7] -> M123/1(CT2)
  [in8] -> M123/2(F2)
  [in9] -> M123/3(E2)
  [in10] -> M123/4(MR2)
  [in11] -> M123/5(T2)
  [in12] -> M123/6(EB2)
  [in13] -> M123/7(CT3)
  [in14] -> M123/8(F3)
  [in15] -> M123/9(E3)
  [in16] -> M123/10(MR3)
  [in17] -> M123/11(T3)
  [in18] -> M123/12(EB3)
  M123/1(LL2) -> Eval122/1(In2)
  M123/2(LL3) -> Eval122/2(In3)
  Eval122/1(Out1) -> To Workspace122/1
  [in7] -> M124/1(CT2)
  [in8] -> M124/2(F2)
  [in9] -> M124/3(E2)
  [in10] -> M124/4(MR2)
  [in11] -> M124/5(T2)
  [in12] -> M124/6(EB2)
  [in13] -> M124/7(CT3)
  [in14] -> M124/8(F3)
  [in15] -> M124/9(E3)
  [in16] -> M124/10(MR3)
  [in17] -> M124/11(T3)
  [in18] -> M124/12(EB3)
  M124/1(LL2) -> Eval123/1(In2)
  M124/2(LL3) -> Eval123/2(In3)
  Eval123/1(Out1) -> To Workspace123/1
  [in7] -> M125/1(CT2)
  [in8] -> M125/2(F2)
  [in9] -> M125/3(E2)
  [in10] -> M125/4(MR2)
  [in11] -> M125/5(T2)
  [in12] -> M125/6(EB2)
  [in13] -> M125/7(CT3)
  [in14] -> M125/8(F3)
  [in15] -> M125/9(E3)
  [in16] -> M125/10(MR3)
  [in17] -> M125/11(T3)
  [in18] -> M125/12(EB3)
  M125/1(LL2) -> Eval124/1(In2)
  M125/2(LL3) -> Eval124/2(In3)
  Eval124/1(Out1) -> To Workspace124/1
  [in7] -> M126/1(CT2)
  [in8] -> M126/2(F2)
  [in9] -> M126/3(E2)
  [in10] -> M126/4(MR2)
  [in11] -> M126/5(T2)
  [in12] -> M126/6(EB2)
  [in13] -> M126/7(CT3)
  [in14] -> M126/8(F3)
  [in15] -> M126/9(E3)
  [in16] -> M126/10(MR3)
  [in17] -> M126/11(T3)
  [in18] -> M126/12(EB3)
  M126/1(LL2) -> Eval125/1(In2)
  M126/2(LL3) -> Eval125/2(In3)
  Eval125/1(Out1) -> To Workspace125/1
  [in7] -> M127/1(CT2)
  [in8] -> M127/2(F2)
  [in9] -> M127/3(E2)
  [in10] -> M127/4(MR2)
  [in11] -> M127/5(T2)
  [in12] -> M127/6(EB2)
  [in13] -> M127/7(CT3)
  [in14] -> M127/8(F3)
  [in15] -> M127/9(E3)
  [in16] -> M127/10(MR3)
  [in17] -> M127/11(T3)
  [in18] -> M127/12(EB3)
  M127/1(LL2) -> Eval126/1(In2)
  M127/2(LL3) -> Eval126/2(In3)
  Eval126/1(Out1) -> To Workspace126/1
  [in7] -> M128/1(CT2)
  [in8] -> M128/2(F2)
  [in9] -> M128/3(E2)
  [in10] -> M128/4(MR2)
  [in11] -> M128/5(T2)
  [in12] -> M128/6(EB2)
  [in13] -> M128/7(CT3)
  [in14] -> M128/8(F3)
  [in15] -> M128/9(E3)
  [in16] -> M128/10(MR3)
  [in17] -> M128/11(T3)
  [in18] -> M128/12(EB3)
  M128/1(LL2) -> Eval127/1(In2)
  M128/2(LL3) -> Eval127/2(In3)
  Eval127/1(Out1) -> To Workspace127/1
  [in7] -> M129/1(CT2)
  [in8] -> M129/2(F2)
  [in9] -> M129/3(E2)
  [in10] -> M129/4(MR2)
  [in11] -> M129/5(T2)
  [in12] -> M129/6(EB2)
  [in13] -> M129/7(CT3)
  [in14] -> M129/8(F3)
  [in15] -> M129/9(E3)
  [in16] -> M129/10(MR3)
  [in17] -> M129/11(T3)
  [in18] -> M129/12(EB3)
  M129/1(LL2) -> Eval128/1(In2)
  M129/2(LL3) -> Eval128/2(In3)
  Eval128/1(Out1) -> To Workspace128/1
  [in7] -> M130/1(CT2)
  [in8] -> M130/2(F2)
  [in9] -> M130/3(E2)
  [in10] -> M130/4(MR2)
  [in11] -> M130/5(T2)
  [in12] -> M130/6(EB2)
  [in13] -> M130/7(CT3)
  [in14] -> M130/8(F3)
  [in15] -> M130/9(E3)
  [in16] -> M130/10(MR3)
  [in17] -> M130/11(T3)
  [in18] -> M130/12(EB3)
  M130/1(LL2) -> Eval129/1(In2)
  M130/2(LL3) -> Eval129/2(In3)
  Eval129/1(Out1) -> To Workspace129/1
  [in7] -> M131/1(CT2)
  [in8] -> M131/2(F2)
  [in9] -> M131/3(E2)
  [in10] -> M131/4(MR2)
  [in11] -> M131/5(T2)
  [in12] -> M131/6(EB2)
  [in13] -> M131/7(CT3)
  [in14] -> M131/8(F3)
  [in15] -> M131/9(E3)
  [in16] -> M131/10(MR3)
  [in17] -> M131/11(T3)
  [in18] -> M131/12(EB3)
  M131/1(LL2) -> Eval130/1(In2)
  M131/2(LL3) -> Eval130/2(In3)
  Eval130/1(Out1) -> To Workspace130/1
  [in7] -> M132/1(CT2)
  [in8] -> M132/2(F2)
  [in9] -> M132/3(E2)
  [in10] -> M132/4(MR2)
  [in11] -> M132/5(T2)
  [in12] -> M132/6(EB2)
  [in13] -> M132/7(CT3)
  [in14] -> M132/8(F3)
  [in15] -> M132/9(E3)
  [in16] -> M132/10(MR3)
  [in17] -> M132/11(T3)
  [in18] -> M132/12(EB3)
  M132/1(LL2) -> Eval131/1(In2)
  M132/2(LL3) -> Eval131/2(In3)
  Eval131/1(Out1) -> To Workspace131/1
  [in7] -> M133/1(CT2)
  [in8] -> M133/2(F2)
  [in9] -> M133/3(E2)
  [in10] -> M133/4(MR2)
  [in11] -> M133/5(T2)
  [in12] -> M133/6(EB2)
  [in13] -> M133/7(CT3)
  [in14] -> M133/8(F3)
  [in15] -> M133/9(E3)
  [in16] -> M133/10(MR3)
  [in17] -> M133/11(T3)
  [in18] -> M133/12(EB3)
  M133/1(LL2) -> Eval132/1(In2)
  M133/2(LL3) -> Eval132/2(In3)
  Eval132/1(Out1) -> To Workspace132/1
  [in7] -> M134/1(CT2)
  [in8] -> M134/2(F2)
  [in9] -> M134/3(E2)
  [in10] -> M134/4(MR2)
  [in11] -> M134/5(T2)
  [in12] -> M134/6(EB2)
  [in13] -> M134/7(CT3)
  [in14] -> M134/8(F3)
  [in15] -> M134/9(E3)
  [in16] -> M134/10(MR3)
  [in17] -> M134/11(T3)
  [in18] -> M134/12(EB3)
  M134/1(LL2) -> Eval133/1(In2)
  M134/2(LL3) -> Eval133/2(In3)
  Eval133/1(Out1) -> To Workspace133/1
  [in7] -> M135/1(CT2)
  [in8] -> M135/2(F2)
  [in9] -> M135/3(E2)
  [in10] -> M135/4(MR2)
  [in11] -> M135/5(T2)
  [in12] -> M135/6(EB2)
  [in13] -> M135/7(CT3)
  [in14] -> M135/8(F3)
  [in15] -> M135/9(E3)
  [in16] -> M135/10(MR3)
  [in17] -> M135/11(T3)
  [in18] -> M135/12(EB3)
  M135/1(LL2) -> Eval134/1(In2)
  M135/2(LL3) -> Eval134/2(In3)
  Eval134/1(Out1) -> To Workspace134/1
  [in7] -> M136/1(CT2)
  [in8] -> M136/2(F2)
  [in9] -> M136/3(E2)
  [in10] -> M136/4(MR2)
  [in11] -> M136/5(T2)
  [in12] -> M136/6(EB2)
  [in13] -> M136/7(CT3)
  [in14] -> M136/8(F3)
  [in15] -> M136/9(E3)
  [in16] -> M136/10(MR3)
  [in17] -> M136/11(T3)
  [in18] -> M136/12(EB3)
  M136/1(LL2) -> Eval135/1(In2)
  M136/2(LL3) -> Eval135/2(In3)
  Eval135/1(Out1) -> To Workspace135/1
  [in7] -> M137/1(CT2)
  [in8] -> M137/2(F2)
  [in9] -> M137/3(E2)
  [in10] -> M137/4(MR2)
  [in11] -> M137/5(T2)
  [in12] -> M137/6(EB2)
  [in13] -> M137/7(CT3)
  [in14] -> M137/8(F3)
  [in15] -> M137/9(E3)
  [in16] -> M137/10(MR3)
  [in17] -> M137/11(T3)
  [in18] -> M137/12(EB3)
  M137/1(LL2) -> Eval136/1(In2)
  M137/2(LL3) -> Eval136/2(In3)
  Eval136/1(Out1) -> To Workspace136/1
  [in7] -> M138/1(CT2)
  [in8] -> M138/2(F2)
  [in9] -> M138/3(E2)
  [in10] -> M138/4(MR2)
  [in11] -> M138/5(T2)
  [in12] -> M138/6(EB2)
  [in13] -> M138/7(CT3)
  [in14] -> M138/8(F3)
  [in15] -> M138/9(E3)
  [in16] -> M138/10(MR3)
  [in17] -> M138/11(T3)
  [in18] -> M138/12(EB3)
  M138/1(LL2) -> Eval137/1(In2)
  M138/2(LL3) -> Eval137/2(In3)
  Eval137/1(Out1) -> To Workspace137/1
  [in7] -> M139/1(CT2)
  [in8] -> M139/2(F2)
  [in9] -> M139/3(E2)
  [in10] -> M139/4(MR2)
  [in11] -> M139/5(T2)
  [in12] -> M139/6(EB2)
  [in13] -> M139/7(CT3)
  [in14] -> M139/8(F3)
  [in15] -> M139/9(E3)
  [in16] -> M139/10(MR3)
  [in17] -> M139/11(T3)
  [in18] -> M139/12(EB3)
  M139/1(LL2) -> Eval138/1(In2)
  M139/2(LL3) -> Eval138/2(In3)
  Eval138/1(Out1) -> To Workspace138/1
  [in7] -> M140/1(CT2)
  [in8] -> M140/2(F2)
  [in9] -> M140/3(E2)
  [in10] -> M140/4(MR2)
  [in11] -> M140/5(T2)
  [in12] -> M140/6(EB2)
  [in13] -> M140/7(CT3)
  [in14] -> M140/8(F3)
  [in15] -> M140/9(E3)
  [in16] -> M140/10(MR3)
  [in17] -> M140/11(T3)
  [in18] -> M140/12(EB3)
  M140/1(LL2) -> Eval139/1(In2)
  M140/2(LL3) -> Eval139/2(In3)
  Eval139/1(Out1) -> To Workspace139/1
  [in7] -> M141/1(CT2)
  [in8] -> M141/2(F2)
  [in9] -> M141/3(E2)
  [in10] -> M141/4(MR2)
  [in11] -> M141/5(T2)
  [in12] -> M141/6(EB2)
  [in13] -> M141/7(CT3)
  [in14] -> M141/8(F3)
  [in15] -> M141/9(E3)
  [in16] -> M141/10(MR3)
  [in17] -> M141/11(T3)
  [in18] -> M141/12(EB3)
  M141/1(LL2) -> Eval140/1(In2)
  M141/2(LL3) -> Eval140/2(In3)
  Eval140/1(Out1) -> To Workspace140/1
  [in7] -> M142/1(CT2)
  [in8] -> M142/2(F2)
  [in9] -> M142/3(E2)
  [in10] -> M142/4(MR2)
  [in11] -> M142/5(T2)
  [in12] -> M142/6(EB2)
  [in13] -> M142/7(CT3)
  [in14] -> M142/8(F3)
  [in15] -> M142/9(E3)
  [in16] -> M142/10(MR3)
  [in17] -> M142/11(T3)
  [in18] -> M142/12(EB3)
  M142/1(LL2) -> Eval141/1(In2)
  M142/2(LL3) -> Eval141/2(In3)
  Eval141/1(Out1) -> To Workspace141/1
  [in7] -> M143/1(CT2)
  [in8] -> M143/2(F2)
  [in9] -> M143/3(E2)
  [in10] -> M143/4(MR2)
  [in11] -> M143/5(T2)
  [in12] -> M143/6(EB2)
  [in13] -> M143/7(CT3)
  [in14] -> M143/8(F3)
  [in15] -> M143/9(E3)
  [in16] -> M143/10(MR3)
  [in17] -> M143/11(T3)
  [in18] -> M143/12(EB3)
  M143/1(LL2) -> Eval142/1(In2)
  M143/2(LL3) -> Eval142/2(In3)
  Eval142/1(Out1) -> To Workspace142/1
  [in7] -> M144/1(CT2)
  [in8] -> M144/2(F2)
  [in9] -> M144/3(E2)
  [in10] -> M144/4(MR2)
  [in11] -> M144/5(T2)
  [in12] -> M144/6(EB2)
  [in13] -> M144/7(CT3)
  [in14] -> M144/8(F3)
  [in15] -> M144/9(E3)
  [in16] -> M144/10(MR3)
  [in17] -> M144/11(T3)
  [in18] -> M144/12(EB3)
  M144/1(LL2) -> Eval143/1(In2)
  M144/2(LL3) -> Eval143/2(In3)
  Eval143/1(Out1) -> To Workspace143/1
  [in7] -> M145/1(CT2)
  [in8] -> M145/2(F2)
  [in9] -> M145/3(E2)
  [in10] -> M145/4(MR2)
  [in11] -> M145/5(T2)
  [in12] -> M145/6(EB2)
  [in13] -> M145/7(CT3)
  [in14] -> M145/8(F3)
  [in15] -> M145/9(E3)
  [in16] -> M145/10(MR3)
  [in17] -> M145/11(T3)
  [in18] -> M145/12(EB3)
  M145/1(LL2) -> Eval144/1(In2)
  M145/2(LL3) -> Eval144/2(In3)
  Eval144/1(Out1) -> To Workspace144/1
  [in7] -> M146/1(CT2)
  [in8] -> M146/2(F2)
  [in9] -> M146/3(E2)
  [in10] -> M146/4(MR2)
  [in11] -> M146/5(T2)
  [in12] -> M146/6(EB2)
  [in13] -> M146/7(CT3)
  [in14] -> M146/8(F3)
  [in15] -> M146/9(E3)
  [in16] -> M146/10(MR3)
  [in17] -> M146/11(T3)
  [in18] -> M146/12(EB3)
  M146/1(LL2) -> Eval145/1(In2)
  M146/2(LL3) -> Eval145/2(In3)
  Eval145/1(Out1) -> To Workspace145/1
  [in7] -> M147/1(CT2)
  [in8] -> M147/2(F2)
  [in9] -> M147/3(E2)
  [in10] -> M147/4(MR2)
  [in11] -> M147/5(T2)
  [in12] -> M147/6(EB2)
  [in13] -> M147/7(CT3)
  [in14] -> M147/8(F3)
  [in15] -> M147/9(E3)
  [in16] -> M147/10(MR3)
  [in17] -> M147/11(T3)
  [in18] -> M147/12(EB3)
  M147/1(LL2) -> Eval146/1(In2)
  M147/2(LL3) -> Eval146/2(In3)
  Eval146/1(Out1) -> To Workspace146/1
  [in7] -> M148/1(CT2)
  [in8] -> M148/2(F2)
  [in9] -> M148/3(E2)
  [in10] -> M148/4(MR2)
  [in11] -> M148/5(T2)
  [in12] -> M148/6(EB2)
  [in13] -> M148/7(CT3)
  [in14] -> M148/8(F3)
  [in15] -> M148/9(E3)
  [in16] -> M148/10(MR3)
  [in17] -> M148/11(T3)
  [in18] -> M148/12(EB3)
  M148/1(LL2) -> Eval147/1(In2)
  M148/2(LL3) -> Eval147/2(In3)
  Eval147/1(Out1) -> To Workspace147/1
  [in7] -> M149/1(CT2)
  [in8] -> M149/2(F2)
  [in9] -> M149/3(E2)
  [in10] -> M149/4(MR2)
  [in11] -> M149/5(T2)
  [in12] -> M149/6(EB2)
  [in13] -> M149/7(CT3)
  [in14] -> M149/8(F3)
  [in15] -> M149/9(E3)
  [in16] -> M149/10(MR3)
  [in17] -> M149/11(T3)
  [in18] -> M149/12(EB3)
  M149/1(LL2) -> Eval148/1(In2)
  M149/2(LL3) -> Eval148/2(In3)
  Eval148/1(Out1) -> To Workspace148/1
  [in7] -> M150/1(CT2)
  [in8] -> M150/2(F2)
  [in9] -> M150/3(E2)
  [in10] -> M150/4(MR2)
  [in11] -> M150/5(T2)
  [in12] -> M150/6(EB2)
  [in13] -> M150/7(CT3)
  [in14] -> M150/8(F3)
  [in15] -> M150/9(E3)
  [in16] -> M150/10(MR3)
  [in17] -> M150/11(T3)
  [in18] -> M150/12(EB3)
  M150/1(LL2) -> Eval149/1(In2)
  M150/2(LL3) -> Eval149/2(In3)
  Eval149/1(Out1) -> To Workspace149/1
  [in7] -> M151/1(CT2)
  [in8] -> M151/2(F2)
  [in9] -> M151/3(E2)
  [in10] -> M151/4(MR2)
  [in11] -> M151/5(T2)
  [in12] -> M151/6(EB2)
  [in13] -> M151/7(CT3)
  [in14] -> M151/8(F3)
  [in15] -> M151/9(E3)
  [in16] -> M151/10(MR3)
  [in17] -> M151/11(T3)
  [in18] -> M151/12(EB3)
  M151/1(LL2) -> Eval150/1(In2)
  M151/2(LL3) -> Eval150/2(In3)
  Eval150/1(Out1) -> To Workspace150/1
  [in7] -> M152/1(CT2)
  [in8] -> M152/2(F2)
  [in9] -> M152/3(E2)
  [in10] -> M152/4(MR2)
  [in11] -> M152/5(T2)
  [in12] -> M152/6(EB2)
  [in13] -> M152/7(CT3)
  [in14] -> M152/8(F3)
  [in15] -> M152/9(E3)
  [in16] -> M152/10(MR3)
  [in17] -> M152/11(T3)
  [in18] -> M152/12(EB3)
  M152/1(LL2) -> Eval151/1(In2)
  M152/2(LL3) -> Eval151/2(In3)
  Eval151/1(Out1) -> To Workspace151/1
  [in7] -> M153/1(CT2)
  [in8] -> M153/2(F2)
  [in9] -> M153/3(E2)
  [in10] -> M153/4(MR2)
  [in11] -> M153/5(T2)
  [in12] -> M153/6(EB2)
  [in13] -> M153/7(CT3)
  [in14] -> M153/8(F3)
  [in15] -> M153/9(E3)
  [in16] -> M153/10(MR3)
  [in17] -> M153/11(T3)
  [in18] -> M153/12(EB3)
  M153/1(LL2) -> Eval152/1(In2)
  M153/2(LL3) -> Eval152/2(In3)
  Eval152/1(Out1) -> To Workspace152/1
  [in7] -> M154/1(CT2)
  [in8] -> M154/2(F2)
  [in9] -> M154/3(E2)
  [in10] -> M154/4(MR2)
  [in11] -> M154/5(T2)
  [in12] -> M154/6(EB2)
  [in13] -> M154/7(CT3)
  [in14] -> M154/8(F3)
  [in15] -> M154/9(E3)
  [in16] -> M154/10(MR3)
  [in17] -> M154/11(T3)
  [in18] -> M154/12(EB3)
  M154/1(LL2) -> Eval153/1(In2)
  M154/2(LL3) -> Eval153/2(In3)
  Eval153/1(Out1) -> To Workspace153/1
  [in7] -> M155/1(CT2)
  [in8] -> M155/2(F2)
  [in9] -> M155/3(E2)
  [in10] -> M155/4(MR2)
  [in11] -> M155/5(T2)
  [in12] -> M155/6(EB2)
  [in13] -> M155/7(CT3)
  [in14] -> M155/8(F3)
  [in15] -> M155/9(E3)
  [in16] -> M155/10(MR3)
  [in17] -> M155/11(T3)
  [in18] -> M155/12(EB3)
  M155/1(LL2) -> Eval154/1(In2)
  M155/2(LL3) -> Eval154/2(In3)
  Eval154/1(Out1) -> To Workspace154/1
  [in7] -> M156/1(CT2)
  [in8] -> M156/2(F2)
  [in9] -> M156/3(E2)
  [in10] -> M156/4(MR2)
  [in11] -> M156/5(T2)
  [in12] -> M156/6(EB2)
  [in13] -> M156/7(CT3)
  [in14] -> M156/8(F3)
  [in15] -> M156/9(E3)
  [in16] -> M156/10(MR3)
  [in17] -> M156/11(T3)
  [in18] -> M156/12(EB3)
  M156/1(LL2) -> Eval155/1(In2)
  M156/2(LL3) -> Eval155/2(In3)
  Eval155/1(Out1) -> To Workspace155/1
  [in7] -> M157/1(CT2)
  [in8] -> M157/2(F2)
  [in9] -> M157/3(E2)
  [in10] -> M157/4(MR2)
  [in11] -> M157/5(T2)
  [in12] -> M157/6(EB2)
  [in13] -> M157/7(CT3)
  [in14] -> M157/8(F3)
  [in15] -> M157/9(E3)
  [in16] -> M157/10(MR3)
  [in17] -> M157/11(T3)
  [in18] -> M157/12(EB3)
  M157/1(LL2) -> Eval156/1(In2)
  M157/2(LL3) -> Eval156/2(In3)
  Eval156/1(Out1) -> To Workspace156/1
  [in7] -> M158/1(CT2)
  [in8] -> M158/2(F2)
  [in9] -> M158/3(E2)
  [in10] -> M158/4(MR2)
  [in11] -> M158/5(T2)
  [in12] -> M158/6(EB2)
  [in13] -> M158/7(CT3)
  [in14] -> M158/8(F3)
  [in15] -> M158/9(E3)
  [in16] -> M158/10(MR3)
  [in17] -> M158/11(T3)
  [in18] -> M158/12(EB3)
  M158/1(LL2) -> Eval157/1(In2)
  M158/2(LL3) -> Eval157/2(In3)
  Eval157/1(Out1) -> To Workspace157/1
  [in7] -> M159/1(CT2)
  [in8] -> M159/2(F2)
  [in9] -> M159/3(E2)
  [in10] -> M159/4(MR2)
  [in11] -> M159/5(T2)
  [in12] -> M159/6(EB2)
  [in13] -> M159/7(CT3)
  [in14] -> M159/8(F3)
  [in15] -> M159/9(E3)
  [in16] -> M159/10(MR3)
  [in17] -> M159/11(T3)
  [in18] -> M159/12(EB3)
  M159/1(LL2) -> Eval158/1(In2)
  M159/2(LL3) -> Eval158/2(In3)
  Eval158/1(Out1) -> To Workspace158/1
  [in7] -> M160/1(CT2)
  [in8] -> M160/2(F2)
  [in9] -> M160/3(E2)
  [in10] -> M160/4(MR2)
  [in11] -> M160/5(T2)
  [in12] -> M160/6(EB2)
  [in13] -> M160/7(CT3)
  [in14] -> M160/8(F3)
  [in15] -> M160/9(E3)
  [in16] -> M160/10(MR3)
  [in17] -> M160/11(T3)
  [in18] -> M160/12(EB3)
  M160/1(LL2) -> Eval159/1(In2)
  M160/2(LL3) -> Eval159/2(In3)
  Eval159/1(Out1) -> To Workspace159/1
  [in7] -> M161/1(CT2)
  [in8] -> M161/2(F2)
  [in9] -> M161/3(E2)
  [in10] -> M161/4(MR2)
  [in11] -> M161/5(T2)
  [in12] -> M161/6(EB2)
  [in13] -> M161/7(CT3)
  [in14] -> M161/8(F3)
  [in15] -> M161/9(E3)
  [in16] -> M161/10(MR3)
  [in17] -> M161/11(T3)
  [in18] -> M161/12(EB3)
  M161/1(LL2) -> Eval160/1(In2)
  M161/2(LL3) -> Eval160/2(In3)
  Eval160/1(Out1) -> To Workspace160/1
  [in7] -> M162/1(CT2)
  [in8] -> M162/2(F2)
  [in9] -> M162/3(E2)
  [in10] -> M162/4(MR2)
  [in11] -> M162/5(T2)
  [in12] -> M162/6(EB2)
  [in13] -> M162/7(CT3)
  [in14] -> M162/8(F3)
  [in15] -> M162/9(E3)
  [in16] -> M162/10(MR3)
  [in17] -> M162/11(T3)
  [in18] -> M162/12(EB3)
  M162/1(LL2) -> Eval161/1(In2)
  M162/2(LL3) -> Eval161/2(In3)
  Eval161/1(Out1) -> To Workspace161/1
  [in7] -> M163/1(CT2)
  [in8] -> M163/2(F2)
  [in9] -> M163/3(E2)
  [in10] -> M163/4(MR2)
  [in11] -> M163/5(T2)
  [in12] -> M163/6(EB2)
  [in13] -> M163/7(CT3)
  [in14] -> M163/8(F3)
  [in15] -> M163/9(E3)
  [in16] -> M163/10(MR3)
  [in17] -> M163/11(T3)
  [in18] -> M163/12(EB3)
  M163/1(LL2) -> Eval162/1(In2)
  M163/2(LL3) -> Eval162/2(In3)
  Eval162/1(Out1) -> To Workspace162/1
  [in7] -> M164/1(CT2)
  [in8] -> M164/2(F2)
  [in9] -> M164/3(E2)
  [in10] -> M164/4(MR2)
  [in11] -> M164/5(T2)
  [in12] -> M164/6(EB2)
  [in13] -> M164/7(CT3)
  [in14] -> M164/8(F3)
  [in15] -> M164/9(E3)
  [in16] -> M164/10(MR3)
  [in17] -> M164/11(T3)
  [in18] -> M164/12(EB3)
  M164/1(LL2) -> Eval163/1(In2)
  M164/2(LL3) -> Eval163/2(In3)
  Eval163/1(Out1) -> To Workspace163/1
  [in7] -> M165/1(CT2)
  [in8] -> M165/2(F2)
  [in9] -> M165/3(E2)
  [in10] -> M165/4(MR2)
  [in11] -> M165/5(T2)
  [in12] -> M165/6(EB2)
  [in13] -> M165/7(CT3)
  [in14] -> M165/8(F3)
  [in15] -> M165/9(E3)
  [in16] -> M165/10(MR3)
  [in17] -> M165/11(T3)
  [in18] -> M165/12(EB3)
  M165/1(LL2) -> Eval164/1(In2)
  M165/2(LL3) -> Eval164/2(In3)
  Eval164/1(Out1) -> To Workspace164/1
  [in7] -> M166/1(CT2)
  [in8] -> M166/2(F2)
  [in9] -> M166/3(E2)
  [in10] -> M166/4(MR2)
  [in11] -> M166/5(T2)
  [in12] -> M166/6(EB2)
  [in13] -> M166/7(CT3)
  [in14] -> M166/8(F3)
  [in15] -> M166/9(E3)
  [in16] -> M166/10(MR3)
  [in17] -> M166/11(T3)
  [in18] -> M166/12(EB3)
  M166/1(LL2) -> Eval165/1(In2)
  M166/2(LL3) -> Eval165/2(In3)
  Eval165/1(Out1) -> To Workspace165/1
  [in7] -> M167/1(CT2)
  [in8] -> M167/2(F2)
  [in9] -> M167/3(E2)
  [in10] -> M167/4(MR2)
  [in11] -> M167/5(T2)
  [in12] -> M167/6(EB2)
  [in13] -> M167/7(CT3)
  [in14] -> M167/8(F3)
  [in15] -> M167/9(E3)
  [in16] -> M167/10(MR3)
  [in17] -> M167/11(T3)
  [in18] -> M167/12(EB3)
  M167/1(LL2) -> Eval166/1(In2)
  M167/2(LL3) -> Eval166/2(In3)
  Eval166/1(Out1) -> To Workspace166/1
  [in7] -> M168/1(CT2)
  [in8] -> M168/2(F2)
  [in9] -> M168/3(E2)
  [in10] -> M168/4(MR2)
  [in11] -> M168/5(T2)
  [in12] -> M168/6(EB2)
  [in13] -> M168/7(CT3)
  [in14] -> M168/8(F3)
  [in15] -> M168/9(E3)
  [in16] -> M168/10(MR3)
  [in17] -> M168/11(T3)
  [in18] -> M168/12(EB3)
  M168/1(LL2) -> Eval167/1(In2)
  M168/2(LL3) -> Eval167/2(In3)
  Eval167/1(Out1) -> To Workspace167/1
  [in7] -> M169/1(CT2)
  [in8] -> M169/2(F2)
  [in9] -> M169/3(E2)
  [in10] -> M169/4(MR2)
  [in11] -> M169/5(T2)
  [in12] -> M169/6(EB2)
  [in13] -> M169/7(CT3)
  [in14] -> M169/8(F3)
  [in15] -> M169/9(E3)
  [in16] -> M169/10(MR3)
  [in17] -> M169/11(T3)
  [in18] -> M169/12(EB3)
  M169/1(LL2) -> Eval168/1(In2)
  M169/2(LL3) -> Eval168/2(In3)
  Eval168/1(Out1) -> To Workspace168/1
  [in7] -> M170/1(CT2)
  [in8] -> M170/2(F2)
  [in9] -> M170/3(E2)
  [in10] -> M170/4(MR2)
  [in11] -> M170/5(T2)
  [in12] -> M170/6(EB2)
  [in13] -> M170/7(CT3)
  [in14] -> M170/8(F3)
  [in15] -> M170/9(E3)
  [in16] -> M170/10(MR3)
  [in17] -> M170/11(T3)
  [in18] -> M170/12(EB3)
  M170/1(LL2) -> Eval169/1(In2)
  M170/2(LL3) -> Eval169/2(In3)
  Eval169/1(Out1) -> To Workspace169/1
  [in7] -> M171/1(CT2)
  [in8] -> M171/2(F2)
  [in9] -> M171/3(E2)
  [in10] -> M171/4(MR2)
  [in11] -> M171/5(T2)
  [in12] -> M171/6(EB2)
  [in13] -> M171/7(CT3)
  [in14] -> M171/8(F3)
  [in15] -> M171/9(E3)
  [in16] -> M171/10(MR3)
  [in17] -> M171/11(T3)
  [in18] -> M171/12(EB3)
  M171/1(LL2) -> Eval170/1(In2)
  M171/2(LL3) -> Eval170/2(In3)
  Eval170/1(Out1) -> To Workspace170/1
  [in7] -> M172/1(CT2)
  [in8] -> M172/2(F2)
  [in9] -> M172/3(E2)
  [in10] -> M172/4(MR2)
  [in11] -> M172/5(T2)
  [in12] -> M172/6(EB2)
  [in13] -> M172/7(CT3)
  [in14] -> M172/8(F3)
  [in15] -> M172/9(E3)
  [in16] -> M172/10(MR3)
  [in17] -> M172/11(T3)
  [in18] -> M172/12(EB3)
  M172/1(LL2) -> Eval171/1(In2)
  M172/2(LL3) -> Eval171/2(In3)
  Eval171/1(Out1) -> To Workspace171/1
  [in7] -> M173/1(CT2)
  [in8] -> M173/2(F2)
  [in9] -> M173/3(E2)
  [in10] -> M173/4(MR2)
  [in11] -> M173/5(T2)
  [in12] -> M173/6(EB2)
  [in13] -> M173/7(CT3)
  [in14] -> M173/8(F3)
  [in15] -> M173/9(E3)
  [in16] -> M173/10(MR3)
  [in17] -> M173/11(T3)
  [in18] -> M173/12(EB3)
  M173/1(LL2) -> Eval172/1(In2)
  M173/2(LL3) -> Eval172/2(In3)
  Eval172/1(Out1) -> To Workspace172/1
  [in7] -> M174/1(CT2)
  [in8] -> M174/2(F2)
  [in9] -> M174/3(E2)
  [in10] -> M174/4(MR2)
  [in11] -> M174/5(T2)
  [in12] -> M174/6(EB2)
  [in13] -> M174/7(CT3)
  [in14] -> M174/8(F3)
  [in15] -> M174/9(E3)
  [in16] -> M174/10(MR3)
  [in17] -> M174/11(T3)
  [in18] -> M174/12(EB3)
  M174/1(LL2) -> Eval173/1(In2)
  M174/2(LL3) -> Eval173/2(In3)
  Eval173/1(Out1) -> To Workspace173/1
  [in7] -> M175/1(CT2)
  [in8] -> M175/2(F2)
  [in9] -> M175/3(E2)
  [in10] -> M175/4(MR2)
  [in11] -> M175/5(T2)
  [in12] -> M175/6(EB2)
  [in13] -> M175/7(CT3)
  [in14] -> M175/8(F3)
  [in15] -> M175/9(E3)
  [in16] -> M175/10(MR3)
  [in17] -> M175/11(T3)
  [in18] -> M175/12(EB3)
  M175/1(LL2) -> Eval174/1(In2)
  M175/2(LL3) -> Eval174/2(In3)
  Eval174/1(Out1) -> To Workspace174/1
  [in7] -> M176/1(CT2)
  [in8] -> M176/2(F2)
  [in9] -> M176/3(E2)
  [in10] -> M176/4(MR2)
  [in11] -> M176/5(T2)
  [in12] -> M176/6(EB2)
  [in13] -> M176/7(CT3)
  [in14] -> M176/8(F3)
  [in15] -> M176/9(E3)
  [in16] -> M176/10(MR3)
  [in17] -> M176/11(T3)
  [in18] -> M176/12(EB3)
  M176/1(LL2) -> Eval175/1(In2)
  M176/2(LL3) -> Eval175/2(In3)
  Eval175/1(Out1) -> To Workspace175/1
  [in7] -> M177/1(CT2)
  [in8] -> M177/2(F2)
  [in9] -> M177/3(E2)
  [in10] -> M177/4(MR2)
  [in11] -> M177/5(T2)
  [in12] -> M177/6(EB2)
  [in13] -> M177/7(CT3)
  [in14] -> M177/8(F3)
  [in15] -> M177/9(E3)
  [in16] -> M177/10(MR3)
  [in17] -> M177/11(T3)
  [in18] -> M177/12(EB3)
  M177/1(LL2) -> Eval176/1(In2)
  M177/2(LL3) -> Eval176/2(In3)
  Eval176/1(Out1) -> To Workspace176/1
  [in7] -> M178/1(CT2)
  [in8] -> M178/2(F2)
  [in9] -> M178/3(E2)
  [in10] -> M178/4(MR2)
  [in11] -> M178/5(T2)
  [in12] -> M178/6(EB2)
  [in13] -> M178/7(CT3)
  [in14] -> M178/8(F3)
  [in15] -> M178/9(E3)
  [in16] -> M178/10(MR3)
  [in17] -> M178/11(T3)
  [in18] -> M178/12(EB3)
  M178/1(LL2) -> Eval177/1(In2)
  M178/2(LL3) -> Eval177/2(In3)
  Eval177/1(Out1) -> To Workspace177/1
  [in7] -> M179/1(CT2)
  [in8] -> M179/2(F2)
  [in9] -> M179/3(E2)
  [in10] -> M179/4(MR2)
  [in11] -> M179/5(T2)
  [in12] -> M179/6(EB2)
  [in13] -> M179/7(CT3)
  [in14] -> M179/8(F3)
  [in15] -> M179/9(E3)
  [in16] -> M179/10(MR3)
  [in17] -> M179/11(T3)
  [in18] -> M179/12(EB3)
  M179/1(LL2) -> Eval178/1(In2)
  M179/2(LL3) -> Eval178/2(In3)
  Eval178/1(Out1) -> To Workspace178/1
  [in7] -> M180/1(CT2)
  [in8] -> M180/2(F2)
  [in9] -> M180/3(E2)
  [in10] -> M180/4(MR2)
  [in11] -> M180/5(T2)
  [in12] -> M180/6(EB2)
  [in13] -> M180/7(CT3)
  [in14] -> M180/8(F3)
  [in15] -> M180/9(E3)
  [in16] -> M180/10(MR3)
  [in17] -> M180/11(T3)
  [in18] -> M180/12(EB3)
  M180/1(LL2) -> Eval179/1(In2)
  M180/2(LL3) -> Eval179/2(In3)
  Eval179/1(Out1) -> To Workspace179/1
  [in7] -> M181/1(CT2)
  [in8] -> M181/2(F2)
  [in9] -> M181/3(E2)
  [in10] -> M181/4(MR2)
  [in11] -> M181/5(T2)
  [in12] -> M181/6(EB2)
  [in13] -> M181/7(CT3)
  [in14] -> M181/8(F3)
  [in15] -> M181/9(E3)
  [in16] -> M181/10(MR3)
  [in17] -> M181/11(T3)
  [in18] -> M181/12(EB3)
  M181/1(LL2) -> Eval180/1(In2)
  M181/2(LL3) -> Eval180/2(In3)
  Eval180/1(Out1) -> To Workspace180/1
  [in7] -> M182/1(CT2)
  [in8] -> M182/2(F2)
  [in9] -> M182/3(E2)
  [in10] -> M182/4(MR2)
  [in11] -> M182/5(T2)
  [in12] -> M182/6(EB2)
  [in13] -> M182/7(CT3)
  [in14] -> M182/8(F3)
  [in15] -> M182/9(E3)
  [in16] -> M182/10(MR3)
  [in17] -> M182/11(T3)
  [in18] -> M182/12(EB3)
  M182/1(LL2) -> Eval181/1(In2)
  M182/2(LL3) -> Eval181/2(In3)
  Eval181/1(Out1) -> To Workspace181/1
  [in7] -> M183/1(CT2)
  [in8] -> M183/2(F2)
  [in9] -> M183/3(E2)
  [in10] -> M183/4(MR2)
  [in11] -> M183/5(T2)
  [in12] -> M183/6(EB2)
  [in13] -> M183/7(CT3)
  [in14] -> M183/8(F3)
  [in15] -> M183/9(E3)
  [in16] -> M183/10(MR3)
  [in17] -> M183/11(T3)
  [in18] -> M183/12(EB3)
  M183/1(LL2) -> Eval182/1(In2)
  M183/2(LL3) -> Eval182/2(In3)
  Eval182/1(Out1) -> To Workspace182/1
  [in7] -> M184/1(CT2)
  [in8] -> M184/2(F2)
  [in9] -> M184/3(E2)
  [in10] -> M184/4(MR2)
  [in11] -> M184/5(T2)
  [in12] -> M184/6(EB2)
  [in13] -> M184/7(CT3)
  [in14] -> M184/8(F3)
  [in15] -> M184/9(E3)
  [in16] -> M184/10(MR3)
  [in17] -> M184/11(T3)
  [in18] -> M184/12(EB3)
  M184/1(LL2) -> Eval183/1(In2)
  M184/2(LL3) -> Eval183/2(In3)
  Eval183/1(Out1) -> To Workspace183/1
  [in7] -> M185/1(CT2)
  [in8] -> M185/2(F2)
  [in9] -> M185/3(E2)
  [in10] -> M185/4(MR2)
  [in11] -> M185/5(T2)
  [in12] -> M185/6(EB2)
  [in13] -> M185/7(CT3)
  [in14] -> M185/8(F3)
  [in15] -> M185/9(E3)
  [in16] -> M185/10(MR3)
  [in17] -> M185/11(T3)
  [in18] -> M185/12(EB3)
  M185/1(LL2) -> Eval184/1(In2)
  M185/2(LL3) -> Eval184/2(In3)
  Eval184/1(Out1) -> To Workspace184/1
  [in7] -> M186/1(CT2)
  [in8] -> M186/2(F2)
  [in9] -> M186/3(E2)
  [in10] -> M186/4(MR2)
  [in11] -> M186/5(T2)
  [in12] -> M186/6(EB2)
  [in13] -> M186/7(CT3)
  [in14] -> M186/8(F3)
  [in15] -> M186/9(E3)
  [in16] -> M186/10(MR3)
  [in17] -> M186/11(T3)
  [in18] -> M186/12(EB3)
  M186/1(LL2) -> Eval185/1(In2)
  M186/2(LL3) -> Eval185/2(In3)
  Eval185/1(Out1) -> To Workspace185/1
  [in7] -> M187/1(CT2)
  [in8] -> M187/2(F2)
  [in9] -> M187/3(E2)
  [in10] -> M187/4(MR2)
  [in11] -> M187/5(T2)
  [in12] -> M187/6(EB2)
  [in13] -> M187/7(CT3)
  [in14] -> M187/8(F3)
  [in15] -> M187/9(E3)
  [in16] -> M187/10(MR3)
  [in17] -> M187/11(T3)
  [in18] -> M187/12(EB3)
  M187/1(LL2) -> Eval186/1(In2)
  M187/2(LL3) -> Eval186/2(In3)
  Eval186/1(Out1) -> To Workspace186/1
  [in7] -> M188/1(CT2)
  [in8] -> M188/2(F2)
  [in9] -> M188/3(E2)
  [in10] -> M188/4(MR2)
  [in11] -> M188/5(T2)
  [in12] -> M188/6(EB2)
  [in13] -> M188/7(CT3)
  [in14] -> M188/8(F3)
  [in15] -> M188/9(E3)
  [in16] -> M188/10(MR3)
  [in17] -> M188/11(T3)
  [in18] -> M188/12(EB3)
  M188/1(LL2) -> Eval187/1(In2)
  M188/2(LL3) -> Eval187/2(In3)
  Eval187/1(Out1) -> To Workspace187/1
  [in7] -> M189/1(CT2)
  [in8] -> M189/2(F2)
  [in9] -> M189/3(E2)
  [in10] -> M189/4(MR2)
  [in11] -> M189/5(T2)
  [in12] -> M189/6(EB2)
  [in13] -> M189/7(CT3)
  [in14] -> M189/8(F3)
  [in15] -> M189/9(E3)
  [in16] -> M189/10(MR3)
  [in17] -> M189/11(T3)
  [in18] -> M189/12(EB3)
  M189/1(LL2) -> Eval188/1(In2)
  M189/2(LL3) -> Eval188/2(In3)
  Eval188/1(Out1) -> To Workspace188/1
  [in7] -> M190/1(CT2)
  [in8] -> M190/2(F2)
  [in9] -> M190/3(E2)
  [in10] -> M190/4(MR2)
  [in11] -> M190/5(T2)
  [in12] -> M190/6(EB2)
  [in13] -> M190/7(CT3)
  [in14] -> M190/8(F3)
  [in15] -> M190/9(E3)
  [in16] -> M190/10(MR3)
  [in17] -> M190/11(T3)
  [in18] -> M190/12(EB3)
  M190/1(LL2) -> Eval189/1(In2)
  M190/2(LL3) -> Eval189/2(In3)
  Eval189/1(Out1) -> To Workspace189/1
  [in7] -> M191/1(CT2)
  [in8] -> M191/2(F2)
  [in9] -> M191/3(E2)
  [in10] -> M191/4(MR2)
  [in11] -> M191/5(T2)
  [in12] -> M191/6(EB2)
  [in13] -> M191/7(CT3)
  [in14] -> M191/8(F3)
  [in15] -> M191/9(E3)
  [in16] -> M191/10(MR3)
  [in17] -> M191/11(T3)
  [in18] -> M191/12(EB3)
  M191/1(LL2) -> Eval190/1(In2)
  M191/2(LL3) -> Eval190/2(In3)
  Eval190/1(Out1) -> To Workspace190/1
  [in7] -> M192/1(CT2)
  [in8] -> M192/2(F2)
  [in9] -> M192/3(E2)
  [in10] -> M192/4(MR2)
  [in11] -> M192/5(T2)
  [in12] -> M192/6(EB2)
  [in13] -> M192/7(CT3)
  [in14] -> M192/8(F3)
  [in15] -> M192/9(E3)
  [in16] -> M192/10(MR3)
  [in17] -> M192/11(T3)
  [in18] -> M192/12(EB3)
  M192/1(LL2) -> Eval191/1(In2)
  M192/2(LL3) -> Eval191/2(In3)
  Eval191/1(Out1) -> To Workspace191/1
  [in7] -> M193/1(CT2)
  [in8] -> M193/2(F2)
  [in9] -> M193/3(E2)
  [in10] -> M193/4(MR2)
  [in11] -> M193/5(T2)
  [in12] -> M193/6(EB2)
  [in13] -> M193/7(CT3)
  [in14] -> M193/8(F3)
  [in15] -> M193/9(E3)
  [in16] -> M193/10(MR3)
  [in17] -> M193/11(T3)
  [in18] -> M193/12(EB3)
  M193/1(LL2) -> Eval192/1(In2)
  M193/2(LL3) -> Eval192/2(In3)
  Eval192/1(Out1) -> To Workspace192/1
  [in7] -> M194/1(CT2)
  [in8] -> M194/2(F2)
  [in9] -> M194/3(E2)
  [in10] -> M194/4(MR2)
  [in11] -> M194/5(T2)
  [in12] -> M194/6(EB2)
  [in13] -> M194/7(CT3)
  [in14] -> M194/8(F3)
  [in15] -> M194/9(E3)
  [in16] -> M194/10(MR3)
  [in17] -> M194/11(T3)
  [in18] -> M194/12(EB3)
  M194/1(LL2) -> Eval193/1(In2)
  M194/2(LL3) -> Eval193/2(In3)
  Eval193/1(Out1) -> To Workspace193/1
  [in7] -> M195/1(CT2)
  [in8] -> M195/2(F2)
  [in9] -> M195/3(E2)
  [in10] -> M195/4(MR2)
  [in11] -> M195/5(T2)
  [in12] -> M195/6(EB2)
  [in13] -> M195/7(CT3)
  [in14] -> M195/8(F3)
  [in15] -> M195/9(E3)
  [in16] -> M195/10(MR3)
  [in17] -> M195/11(T3)
  [in18] -> M195/12(EB3)
  M195/1(LL2) -> Eval194/1(In2)
  M195/2(LL3) -> Eval194/2(In3)
  Eval194/1(Out1) -> To Workspace194/1
  [in7] -> M196/1(CT2)
  [in8] -> M196/2(F2)
  [in9] -> M196/3(E2)
  [in10] -> M196/4(MR2)
  [in11] -> M196/5(T2)
  [in12] -> M196/6(EB2)
  [in13] -> M196/7(CT3)
  [in14] -> M196/8(F3)
  [in15] -> M196/9(E3)
  [in16] -> M196/10(MR3)
  [in17] -> M196/11(T3)
  [in18] -> M196/12(EB3)
  M196/1(LL2) -> Eval195/1(In2)
  M196/2(LL3) -> Eval195/2(In3)
  Eval195/1(Out1) -> To Workspace195/1
  [in7] -> M197/1(CT2)
  [in8] -> M197/2(F2)
  [in9] -> M197/3(E2)
  [in10] -> M197/4(MR2)
  [in11] -> M197/5(T2)
  [in12] -> M197/6(EB2)
  [in13] -> M197/7(CT3)
  [in14] -> M197/8(F3)
  [in15] -> M197/9(E3)
  [in16] -> M197/10(MR3)
  [in17] -> M197/11(T3)
  [in18] -> M197/12(EB3)
  M197/1(LL2) -> Eval196/1(In2)
  M197/2(LL3) -> Eval196/2(In3)
  Eval196/1(Out1) -> To Workspace196/1
  [in7] -> M198/1(CT2)
  [in8] -> M198/2(F2)
  [in9] -> M198/3(E2)
  [in10] -> M198/4(MR2)
  [in11] -> M198/5(T2)
  [in12] -> M198/6(EB2)
  [in13] -> M198/7(CT3)
  [in14] -> M198/8(F3)
  [in15] -> M198/9(E3)
  [in16] -> M198/10(MR3)
  [in17] -> M198/11(T3)
  [in18] -> M198/12(EB3)
  M198/1(LL2) -> Eval197/1(In2)
  M198/2(LL3) -> Eval197/2(In3)
  Eval197/1(Out1) -> To Workspace197/1
  [in7] -> M199/1(CT2)
  [in8] -> M199/2(F2)
  [in9] -> M199/3(E2)
  [in10] -> M199/4(MR2)
  [in11] -> M199/5(T2)
  [in12] -> M199/6(EB2)
  [in13] -> M199/7(CT3)
  [in14] -> M199/8(F3)
  [in15] -> M199/9(E3)
  [in16] -> M199/10(MR3)
  [in17] -> M199/11(T3)
  [in18] -> M199/12(EB3)
  M199/1(LL2) -> Eval198/1(In2)
  M199/2(LL3) -> Eval198/2(In3)
  Eval198/1(Out1) -> To Workspace198/1
  [in7] -> M200/1(CT2)
  [in8] -> M200/2(F2)
  [in9] -> M200/3(E2)
  [in10] -> M200/4(MR2)
  [in11] -> M200/5(T2)
  [in12] -> M200/6(EB2)
  [in13] -> M200/7(CT3)
  [in14] -> M200/8(F3)
  [in15] -> M200/9(E3)
  [in16] -> M200/10(MR3)
  [in17] -> M200/11(T3)
  [in18] -> M200/12(EB3)
  M200/1(LL2) -> Eval199/1(In2)
  M200/2(LL3) -> Eval199/2(In3)
  Eval199/1(Out1) -> To Workspace199/1
  [in7] -> M201/1(CT2)
  [in8] -> M201/2(F2)
  [in9] -> M201/3(E2)
  [in10] -> M201/4(MR2)
  [in11] -> M201/5(T2)
  [in12] -> M201/6(EB2)
  [in13] -> M201/7(CT3)
  [in14] -> M201/8(F3)
  [in15] -> M201/9(E3)
  [in16] -> M201/10(MR3)
  [in17] -> M201/11(T3)
  [in18] -> M201/12(EB3)
  M201/1(LL2) -> Eval200/1(In2)
  M201/2(LL3) -> Eval200/2(In3)
  Eval200/1(Out1) -> To Workspace200/1
  [in7] -> M202/1(CT2)
  [in8] -> M202/2(F2)
  [in9] -> M202/3(E2)
  [in10] -> M202/4(MR2)
  [in11] -> M202/5(T2)
  [in12] -> M202/6(EB2)
  [in13] -> M202/7(CT3)
  [in14] -> M202/8(F3)
  [in15] -> M202/9(E3)
  [in16] -> M202/10(MR3)
  [in17] -> M202/11(T3)
  [in18] -> M202/12(EB3)
  M202/1(LL2) -> Eval201/1(In2)
  M202/2(LL3) -> Eval201/2(In3)
  Eval201/1(Out1) -> To Workspace201/1
  [in7] -> M203/1(CT2)
  [in8] -> M203/2(F2)
  [in9] -> M203/3(E2)
  [in10] -> M203/4(MR2)
  [in11] -> M203/5(T2)
  [in12] -> M203/6(EB2)
  [in13] -> M203/7(CT3)
  [in14] -> M203/8(F3)
  [in15] -> M203/9(E3)
  [in16] -> M203/10(MR3)
  [in17] -> M203/11(T3)
  [in18] -> M203/12(EB3)
  M203/1(LL2) -> Eval202/1(In2)
  M203/2(LL3) -> Eval202/2(In3)
  Eval202/1(Out1) -> To Workspace202/1
  [in7] -> M204/1(CT2)
  [in8] -> M204/2(F2)
  [in9] -> M204/3(E2)
  [in10] -> M204/4(MR2)
  [in11] -> M204/5(T2)
  [in12] -> M204/6(EB2)
  [in13] -> M204/7(CT3)
  [in14] -> M204/8(F3)
  [in15] -> M204/9(E3)
  [in16] -> M204/10(MR3)
  [in17] -> M204/11(T3)
  [in18] -> M204/12(EB3)
  M204/1(LL2) -> Eval203/1(In2)
  M204/2(LL3) -> Eval203/2(In3)
  Eval203/1(Out1) -> To Workspace203/1
  [in7] -> M205/1(CT2)
  [in8] -> M205/2(F2)
  [in9] -> M205/3(E2)
  [in10] -> M205/4(MR2)
  [in11] -> M205/5(T2)
  [in12] -> M205/6(EB2)
  [in13] -> M205/7(CT3)
  [in14] -> M205/8(F3)
  [in15] -> M205/9(E3)
  [in16] -> M205/10(MR3)
  [in17] -> M205/11(T3)
  [in18] -> M205/12(EB3)
  M205/1(LL2) -> Eval204/1(In2)
  M205/2(LL3) -> Eval204/2(In3)
  Eval204/1(Out1) -> To Workspace204/1
  [in7] -> M206/1(CT2)
  [in8] -> M206/2(F2)
  [in9] -> M206/3(E2)
  [in10] -> M206/4(MR2)
  [in11] -> M206/5(T2)
  [in12] -> M206/6(EB2)
  [in13] -> M206/7(CT3)
  [in14] -> M206/8(F3)
  [in15] -> M206/9(E3)
  [in16] -> M206/10(MR3)
  [in17] -> M206/11(T3)
  [in18] -> M206/12(EB3)
  M206/1(LL2) -> Eval205/1(In2)
  M206/2(LL3) -> Eval205/2(In3)
  Eval205/1(Out1) -> To Workspace205/1
  [in7] -> M207/1(CT2)
  [in8] -> M207/2(F2)
  [in9] -> M207/3(E2)
  [in10] -> M207/4(MR2)
  [in11] -> M207/5(T2)
  [in12] -> M207/6(EB2)
  [in13] -> M207/7(CT3)
  [in14] -> M207/8(F3)
  [in15] -> M207/9(E3)
  [in16] -> M207/10(MR3)
  [in17] -> M207/11(T3)
  [in18] -> M207/12(EB3)
  M207/1(LL2) -> Eval206/1(In2)
  M207/2(LL3) -> Eval206/2(In3)
  Eval206/1(Out1) -> To Workspace206/1
  [in7] -> M208/1(CT2)
  [in8] -> M208/2(F2)
  [in9] -> M208/3(E2)
  [in10] -> M208/4(MR2)
  [in11] -> M208/5(T2)
  [in12] -> M208/6(EB2)
  [in13] -> M208/7(CT3)
  [in14] -> M208/8(F3)
  [in15] -> M208/9(E3)
  [in16] -> M208/10(MR3)
  [in17] -> M208/11(T3)
  [in18] -> M208/12(EB3)
  M208/1(LL2) -> Eval207/1(In2)
  M208/2(LL3) -> Eval207/2(In3)
  Eval207/1(Out1) -> To Workspace207/1
  [in7] -> M209/1(CT2)
  [in8] -> M209/2(F2)
  [in9] -> M209/3(E2)
  [in10] -> M209/4(MR2)
  [in11] -> M209/5(T2)
  [in12] -> M209/6(EB2)
  [in13] -> M209/7(CT3)
  [in14] -> M209/8(F3)
  [in15] -> M209/9(E3)
  [in16] -> M209/10(MR3)
  [in17] -> M209/11(T3)
  [in18] -> M209/12(EB3)
  M209/1(LL2) -> Eval208/1(In2)
  M209/2(LL3) -> Eval208/2(In3)
  Eval208/1(Out1) -> To Workspace208/1
  [in7] -> M210/1(CT2)
  [in8] -> M210/2(F2)
  [in9] -> M210/3(E2)
  [in10] -> M210/4(MR2)
  [in11] -> M210/5(T2)
  [in12] -> M210/6(EB2)
  [in13] -> M210/7(CT3)
  [in14] -> M210/8(F3)
  [in15] -> M210/9(E3)
  [in16] -> M210/10(MR3)
  [in17] -> M210/11(T3)
  [in18] -> M210/12(EB3)
  M210/1(LL2) -> Eval209/1(In2)
  M210/2(LL3) -> Eval209/2(In3)
  Eval209/1(Out1) -> To Workspace209/1
  [in7] -> M211/1(CT2)
  [in8] -> M211/2(F2)
  [in9] -> M211/3(E2)
  [in10] -> M211/4(MR2)
  [in11] -> M211/5(T2)
  [in12] -> M211/6(EB2)
  [in13] -> M211/7(CT3)
  [in14] -> M211/8(F3)
  [in15] -> M211/9(E3)
  [in16] -> M211/10(MR3)
  [in17] -> M211/11(T3)
  [in18] -> M211/12(EB3)
  M211/1(LL2) -> Eval210/1(In2)
  M211/2(LL3) -> Eval210/2(In3)
  Eval210/1(Out1) -> To Workspace210/1
  [in7] -> M212/1(CT2)
  [in8] -> M212/2(F2)
  [in9] -> M212/3(E2)
  [in10] -> M212/4(MR2)
  [in11] -> M212/5(T2)
  [in12] -> M212/6(EB2)
  [in13] -> M212/7(CT3)
  [in14] -> M212/8(F3)
  [in15] -> M212/9(E3)
  [in16] -> M212/10(MR3)
  [in17] -> M212/11(T3)
  [in18] -> M212/12(EB3)
  M212/1(LL2) -> Eval211/1(In2)
  M212/2(LL3) -> Eval211/2(In3)
  Eval211/1(Out1) -> To Workspace211/1
  [in7] -> M213/1(CT2)
  [in8] -> M213/2(F2)
  [in9] -> M213/3(E2)
  [in10] -> M213/4(MR2)
  [in11] -> M213/5(T2)
  [in12] -> M213/6(EB2)
  [in13] -> M213/7(CT3)
  [in14] -> M213/8(F3)
  [in15] -> M213/9(E3)
  [in16] -> M213/10(MR3)
  [in17] -> M213/11(T3)
  [in18] -> M213/12(EB3)
  M213/1(LL2) -> Eval212/1(In2)
  M213/2(LL3) -> Eval212/2(In3)
  Eval212/1(Out1) -> To Workspace212/1
  [in7] -> M214/1(CT2)
  [in8] -> M214/2(F2)
  [in9] -> M214/3(E2)
  [in10] -> M214/4(MR2)
  [in11] -> M214/5(T2)
  [in12] -> M214/6(EB2)
  [in13] -> M214/7(CT3)
  [in14] -> M214/8(F3)
  [in15] -> M214/9(E3)
  [in16] -> M214/10(MR3)
  [in17] -> M214/11(T3)
  [in18] -> M214/12(EB3)
  M214/1(LL2) -> Eval213/1(In2)
  M214/2(LL3) -> Eval213/2(In3)
  Eval213/1(Out1) -> To Workspace213/1
  [in7] -> M215/1(CT2)
  [in8] -> M215/2(F2)
  [in9] -> M215/3(E2)
  [in10] -> M215/4(MR2)
  [in11] -> M215/5(T2)
  [in12] -> M215/6(EB2)
  [in13] -> M215/7(CT3)
  [in14] -> M215/8(F3)
  [in15] -> M215/9(E3)
  [in16] -> M215/10(MR3)
  [in17] -> M215/11(T3)
  [in18] -> M215/12(EB3)
  M215/1(LL2) -> Eval214/1(In2)
  M215/2(LL3) -> Eval214/2(In3)
  Eval214/1(Out1) -> To Workspace214/1
  [in7] -> M216/1(CT2)
  [in8] -> M216/2(F2)
  [in9] -> M216/3(E2)
  [in10] -> M216/4(MR2)
  [in11] -> M216/5(T2)
  [in12] -> M216/6(EB2)
  [in13] -> M216/7(CT3)
  [in14] -> M216/8(F3)
  [in15] -> M216/9(E3)
  [in16] -> M216/10(MR3)
  [in17] -> M216/11(T3)
  [in18] -> M216/12(EB3)
  M216/1(LL2) -> Eval215/1(In2)
  M216/2(LL3) -> Eval215/2(In3)
  Eval215/1(Out1) -> To Workspace215/1
  [in7] -> M217/1(CT2)
  [in8] -> M217/2(F2)
  [in9] -> M217/3(E2)
  [in10] -> M217/4(MR2)
  [in11] -> M217/5(T2)
  [in12] -> M217/6(EB2)
  [in13] -> M217/7(CT3)
  [in14] -> M217/8(F3)
  [in15] -> M217/9(E3)
  [in16] -> M217/10(MR3)
  [in17] -> M217/11(T3)
  [in18] -> M217/12(EB3)
  M217/1(LL2) -> Eval216/1(In2)
  M217/2(LL3) -> Eval216/2(In3)
  Eval216/1(Out1) -> To Workspace216/1
  [in7] -> M218/1(CT2)
  [in8] -> M218/2(F2)
  [in9] -> M218/3(E2)
  [in10] -> M218/4(MR2)
  [in11] -> M218/5(T2)
  [in12] -> M218/6(EB2)
  [in13] -> M218/7(CT3)
  [in14] -> M218/8(F3)
  [in15] -> M218/9(E3)
  [in16] -> M218/10(MR3)
  [in17] -> M218/11(T3)
  [in18] -> M218/12(EB3)
  M218/1(LL2) -> Eval217/1(In2)
  M218/2(LL3) -> Eval217/2(In3)
  Eval217/1(Out1) -> To Workspace217/1
  [in7] -> M219/1(CT2)
  [in8] -> M219/2(F2)
  [in9] -> M219/3(E2)
  [in10] -> M219/4(MR2)
  [in11] -> M219/5(T2)
  [in12] -> M219/6(EB2)
  [in13] -> M219/7(CT3)
  [in14] -> M219/8(F3)
  [in15] -> M219/9(E3)
  [in16] -> M219/10(MR3)
  [in17] -> M219/11(T3)
  [in18] -> M219/12(EB3)
  M219/1(LL2) -> Eval218/1(In2)
  M219/2(LL3) -> Eval218/2(In3)
  Eval218/1(Out1) -> To Workspace218/1
  [in7] -> M220/1(CT2)
  [in8] -> M220/2(F2)
  [in9] -> M220/3(E2)
  [in10] -> M220/4(MR2)
  [in11] -> M220/5(T2)
  [in12] -> M220/6(EB2)
  [in13] -> M220/7(CT3)
  [in14] -> M220/8(F3)
  [in15] -> M220/9(E3)
  [in16] -> M220/10(MR3)
  [in17] -> M220/11(T3)
  [in18] -> M220/12(EB3)
  M220/1(LL2) -> Eval219/1(In2)
  M220/2(LL3) -> Eval219/2(In3)
  Eval219/1(Out1) -> To Workspace219/1
  [in7] -> M221/1(CT2)
  [in8] -> M221/2(F2)
  [in9] -> M221/3(E2)
  [in10] -> M221/4(MR2)
  [in11] -> M221/5(T2)
  [in12] -> M221/6(EB2)
  [in13] -> M221/7(CT3)
  [in14] -> M221/8(F3)
  [in15] -> M221/9(E3)
  [in16] -> M221/10(MR3)
  [in17] -> M221/11(T3)
  [in18] -> M221/12(EB3)
  M221/1(LL2) -> Eval220/1(In2)
  M221/2(LL3) -> Eval220/2(In3)
  Eval220/1(Out1) -> To Workspace220/1
  [in7] -> M222/1(CT2)
  [in8] -> M222/2(F2)
  [in9] -> M222/3(E2)
  [in10] -> M222/4(MR2)
  [in11] -> M222/5(T2)
  [in12] -> M222/6(EB2)
  [in13] -> M222/7(CT3)
  [in14] -> M222/8(F3)
  [in15] -> M222/9(E3)
  [in16] -> M222/10(MR3)
  [in17] -> M222/11(T3)
  [in18] -> M222/12(EB3)
  M222/1(LL2) -> Eval221/1(In2)
  M222/2(LL3) -> Eval221/2(In3)
  Eval221/1(Out1) -> To Workspace221/1
  [in7] -> M223/1(CT2)
  [in8] -> M223/2(F2)
  [in9] -> M223/3(E2)
  [in10] -> M223/4(MR2)
  [in11] -> M223/5(T2)
  [in12] -> M223/6(EB2)
  [in13] -> M223/7(CT3)
  [in14] -> M223/8(F3)
  [in15] -> M223/9(E3)
  [in16] -> M223/10(MR3)
  [in17] -> M223/11(T3)
  [in18] -> M223/12(EB3)
  M223/1(LL2) -> Eval222/1(In2)
  M223/2(LL3) -> Eval222/2(In3)
  Eval222/1(Out1) -> To Workspace222/1
  [in7] -> M224/1(CT2)
  [in8] -> M224/2(F2)
  [in9] -> M224/3(E2)
  [in10] -> M224/4(MR2)
  [in11] -> M224/5(T2)
  [in12] -> M224/6(EB2)
  [in13] -> M224/7(CT3)
  [in14] -> M224/8(F3)
  [in15] -> M224/9(E3)
  [in16] -> M224/10(MR3)
  [in17] -> M224/11(T3)
  [in18] -> M224/12(EB3)
  M224/1(LL2) -> Eval223/1(In2)
  M224/2(LL3) -> Eval223/2(In3)
  Eval223/1(Out1) -> To Workspace223/1
  [in7] -> M225/1(CT2)
  [in8] -> M225/2(F2)
  [in9] -> M225/3(E2)
  [in10] -> M225/4(MR2)
  [in11] -> M225/5(T2)
  [in12] -> M225/6(EB2)
  [in13] -> M225/7(CT3)
  [in14] -> M225/8(F3)
  [in15] -> M225/9(E3)
  [in16] -> M225/10(MR3)
  [in17] -> M225/11(T3)
  [in18] -> M225/12(EB3)
  M225/1(LL2) -> Eval224/1(In2)
  M225/2(LL3) -> Eval224/2(In3)
  Eval224/1(Out1) -> To Workspace224/1
  [in7] -> M226/1(CT2)
  [in8] -> M226/2(F2)
  [in9] -> M226/3(E2)
  [in10] -> M226/4(MR2)
  [in11] -> M226/5(T2)
  [in12] -> M226/6(EB2)
  [in13] -> M226/7(CT3)
  [in14] -> M226/8(F3)
  [in15] -> M226/9(E3)
  [in16] -> M226/10(MR3)
  [in17] -> M226/11(T3)
  [in18] -> M226/12(EB3)
  M226/1(LL2) -> Eval225/1(In2)
  M226/2(LL3) -> Eval225/2(In3)
  Eval225/1(Out1) -> To Workspace225/1
  [in7] -> M227/1(CT2)
  [in8] -> M227/2(F2)
  [in9] -> M227/3(E2)
  [in10] -> M227/4(MR2)
  [in11] -> M227/5(T2)
  [in12] -> M227/6(EB2)
  [in13] -> M227/7(CT3)
  [in14] -> M227/8(F3)
  [in15] -> M227/9(E3)
  [in16] -> M227/10(MR3)
  [in17] -> M227/11(T3)
  [in18] -> M227/12(EB3)
  M227/1(LL2) -> Eval226/1(In2)
  M227/2(LL3) -> Eval226/2(In3)
  Eval226/1(Out1) -> To Workspace226/1
  [in7] -> M228/1(CT2)
  [in8] -> M228/2(F2)
  [in9] -> M228/3(E2)
  [in10] -> M228/4(MR2)
  [in11] -> M228/5(T2)
  [in12] -> M228/6(EB2)
  [in13] -> M228/7(CT3)
  [in14] -> M228/8(F3)
  [in15] -> M228/9(E3)
  [in16] -> M228/10(MR3)
  [in17] -> M228/11(T3)
  [in18] -> M228/12(EB3)
  M228/1(LL2) -> Eval227/1(In2)
  M228/2(LL3) -> Eval227/2(In3)
  Eval227/1(Out1) -> To Workspace227/1
  [in7] -> M229/1(CT2)
  [in8] -> M229/2(F2)
  [in9] -> M229/3(E2)
  [in10] -> M229/4(MR2)
  [in11] -> M229/5(T2)
  [in12] -> M229/6(EB2)
  [in13] -> M229/7(CT3)
  [in14] -> M229/8(F3)
  [in15] -> M229/9(E3)
  [in16] -> M229/10(MR3)
  [in17] -> M229/11(T3)
  [in18] -> M229/12(EB3)
  M229/1(LL2) -> Eval228/1(In2)
  M229/2(LL3) -> Eval228/2(In3)
  Eval228/1(Out1) -> To Workspace228/1
  [in7] -> M230/1(CT2)
  [in8] -> M230/2(F2)
  [in9] -> M230/3(E2)
  [in10] -> M230/4(MR2)
  [in11] -> M230/5(T2)
  [in12] -> M230/6(EB2)
  [in13] -> M230/7(CT3)
  [in14] -> M230/8(F3)
  [in15] -> M230/9(E3)
  [in16] -> M230/10(MR3)
  [in17] -> M230/11(T3)
  [in18] -> M230/12(EB3)
  M230/1(LL2) -> Eval229/1(In2)
  M230/2(LL3) -> Eval229/2(In3)
  Eval229/1(Out1) -> To Workspace229/1
  [in7] -> M231/1(CT2)
  [in8] -> M231/2(F2)
  [in9] -> M231/3(E2)
  [in10] -> M231/4(MR2)
  [in11] -> M231/5(T2)
  [in12] -> M231/6(EB2)
  [in13] -> M231/7(CT3)
  [in14] -> M231/8(F3)
  [in15] -> M231/9(E3)
  [in16] -> M231/10(MR3)
  [in17] -> M231/11(T3)
  [in18] -> M231/12(EB3)
  M231/1(LL2) -> Eval230/1(In2)
  M231/2(LL3) -> Eval230/2(In3)
  Eval230/1(Out1) -> To Workspace230/1
  [in7] -> M232/1(CT2)
  [in8] -> M232/2(F2)
  [in9] -> M232/3(E2)
  [in10] -> M232/4(MR2)
  [in11] -> M232/5(T2)
  [in12] -> M232/6(EB2)
  [in13] -> M232/7(CT3)
  [in14] -> M232/8(F3)
  [in15] -> M232/9(E3)
  [in16] -> M232/10(MR3)
  [in17] -> M232/11(T3)
  [in18] -> M232/12(EB3)
  M232/1(LL2) -> Eval231/1(In2)
  M232/2(LL3) -> Eval231/2(In3)
  Eval231/1(Out1) -> To Workspace231/1
  [in7] -> M233/1(CT2)
  [in8] -> M233/2(F2)
  [in9] -> M233/3(E2)
  [in10] -> M233/4(MR2)
  [in11] -> M233/5(T2)
  [in12] -> M233/6(EB2)
  [in13] -> M233/7(CT3)
  [in14] -> M233/8(F3)
  [in15] -> M233/9(E3)
  [in16] -> M233/10(MR3)
  [in17] -> M233/11(T3)
  [in18] -> M233/12(EB3)
  M233/1(LL2) -> Eval232/1(In2)
  M233/2(LL3) -> Eval232/2(In3)
  Eval232/1(Out1) -> To Workspace232/1
  [in7] -> M234/1(CT2)
  [in8] -> M234/2(F2)
  [in9] -> M234/3(E2)
  [in10] -> M234/4(MR2)
  [in11] -> M234/5(T2)
  [in12] -> M234/6(EB2)
  [in13] -> M234/7(CT3)
  [in14] -> M234/8(F3)
  [in15] -> M234/9(E3)
  [in16] -> M234/10(MR3)
  [in17] -> M234/11(T3)
  [in18] -> M234/12(EB3)
  M234/1(LL2) -> Eval233/1(In2)
  M234/2(LL3) -> Eval233/2(In3)
  Eval233/1(Out1) -> To Workspace233/1
  [in7] -> M235/1(CT2)
  [in8] -> M235/2(F2)
  [in9] -> M235/3(E2)
  [in10] -> M235/4(MR2)
  [in11] -> M235/5(T2)
  [in12] -> M235/6(EB2)
  [in13] -> M235/7(CT3)
  [in14] -> M235/8(F3)
  [in15] -> M235/9(E3)
  [in16] -> M235/10(MR3)
  [in17] -> M235/11(T3)
  [in18] -> M235/12(EB3)
  M235/1(LL2) -> Eval234/1(In2)
  M235/2(LL3) -> Eval234/2(In3)
  Eval234/1(Out1) -> To Workspace234/1
  [in7] -> M236/1(CT2)
  [in8] -> M236/2(F2)
  [in9] -> M236/3(E2)
  [in10] -> M236/4(MR2)
  [in11] -> M236/5(T2)
  [in12] -> M236/6(EB2)
  [in13] -> M236/7(CT3)
  [in14] -> M236/8(F3)
  [in15] -> M236/9(E3)
  [in16] -> M236/10(MR3)
  [in17] -> M236/11(T3)
  [in18] -> M236/12(EB3)
  M236/1(LL2) -> Eval235/1(In2)
  M236/2(LL3) -> Eval235/2(In3)
  Eval235/1(Out1) -> To Workspace235/1
  [in7] -> M237/1(CT2)
  [in8] -> M237/2(F2)
  [in9] -> M237/3(E2)
  [in10] -> M237/4(MR2)
  [in11] -> M237/5(T2)
  [in12] -> M237/6(EB2)
  [in13] -> M237/7(CT3)
  [in14] -> M237/8(F3)
  [in15] -> M237/9(E3)
  [in16] -> M237/10(MR3)
  [in17] -> M237/11(T3)
  [in18] -> M237/12(EB3)
  M237/1(LL2) -> Eval236/1(In2)
  M237/2(LL3) -> Eval236/2(In3)
  Eval236/1(Out1) -> To Workspace236/1
  [in7] -> M238/1(CT2)
  [in8] -> M238/2(F2)
  [in9] -> M238/3(E2)
  [in10] -> M238/4(MR2)
  [in11] -> M238/5(T2)
  [in12] -> M238/6(EB2)
  [in13] -> M238/7(CT3)
  [in14] -> M238/8(F3)
  [in15] -> M238/9(E3)
  [in16] -> M238/10(MR3)
  [in17] -> M238/11(T3)
  [in18] -> M238/12(EB3)
  M238/1(LL2) -> Eval237/1(In2)
  M238/2(LL3) -> Eval237/2(In3)
  Eval237/1(Out1) -> To Workspace237/1
  [in7] -> M239/1(CT2)
  [in8] -> M239/2(F2)
  [in9] -> M239/3(E2)
  [in10] -> M239/4(MR2)
  [in11] -> M239/5(T2)
  [in12] -> M239/6(EB2)
  [in13] -> M239/7(CT3)
  [in14] -> M239/8(F3)
  [in15] -> M239/9(E3)
  [in16] -> M239/10(MR3)
  [in17] -> M239/11(T3)
  [in18] -> M239/12(EB3)
  M239/1(LL2) -> Eval238/1(In2)
  M239/2(LL3) -> Eval238/2(In3)
  Eval238/1(Out1) -> To Workspace238/1
  [in7] -> M240/1(CT2)
  [in8] -> M240/2(F2)
  [in9] -> M240/3(E2)
  [in10] -> M240/4(MR2)
  [in11] -> M240/5(T2)
  [in12] -> M240/6(EB2)
  [in13] -> M240/7(CT3)
  [in14] -> M240/8(F3)
  [in15] -> M240/9(E3)
  [in16] -> M240/10(MR3)
  [in17] -> M240/11(T3)
  [in18] -> M240/12(EB3)
  M240/1(LL2) -> Eval239/1(In2)
  M240/2(LL3) -> Eval239/2(In3)
  Eval239/1(Out1) -> To Workspace239/1
  [in7] -> M241/1(CT2)
  [in8] -> M241/2(F2)
  [in9] -> M241/3(E2)
  [in10] -> M241/4(MR2)
  [in11] -> M241/5(T2)
  [in12] -> M241/6(EB2)
  [in13] -> M241/7(CT3)
  [in14] -> M241/8(F3)
  [in15] -> M241/9(E3)
  [in16] -> M241/10(MR3)
  [in17] -> M241/11(T3)
  [in18] -> M241/12(EB3)
  M241/1(LL2) -> Eval240/1(In2)
  M241/2(LL3) -> Eval240/2(In3)
  Eval240/1(Out1) -> To Workspace240/1
  [in7] -> M242/1(CT2)
  [in8] -> M242/2(F2)
  [in9] -> M242/3(E2)
  [in10] -> M242/4(MR2)
  [in11] -> M242/5(T2)
  [in12] -> M242/6(EB2)
  [in13] -> M242/7(CT3)
  [in14] -> M242/8(F3)
  [in15] -> M242/9(E3)
  [in16] -> M242/10(MR3)
  [in17] -> M242/11(T3)
  [in18] -> M242/12(EB3)
  M242/1(LL2) -> Eval241/1(In2)
  M242/2(LL3) -> Eval241/2(In3)
  Eval241/1(Out1) -> To Workspace241/1
  [in7] -> M243/1(CT2)
  [in8] -> M243/2(F2)
  [in9] -> M243/3(E2)
  [in10] -> M243/4(MR2)
  [in11] -> M243/5(T2)
  [in12] -> M243/6(EB2)
  [in13] -> M243/7(CT3)
  [in14] -> M243/8(F3)
  [in15] -> M243/9(E3)
  [in16] -> M243/10(MR3)
  [in17] -> M243/11(T3)
  [in18] -> M243/12(EB3)
  M243/1(LL2) -> Eval242/1(In2)
  M243/2(LL3) -> Eval242/2(In3)
  Eval242/1(Out1) -> To Workspace242/1
  [in7] -> M244/1(CT2)
  [in8] -> M244/2(F2)
  [in9] -> M244/3(E2)
  [in10] -> M244/4(MR2)
  [in11] -> M244/5(T2)
  [in12] -> M244/6(EB2)
  [in13] -> M244/7(CT3)
  [in14] -> M244/8(F3)
  [in15] -> M244/9(E3)
  [in16] -> M244/10(MR3)
  [in17] -> M244/11(T3)
  [in18] -> M244/12(EB3)
  M244/1(LL2) -> Eval243/1(In2)
  M244/2(LL3) -> Eval243/2(In3)
  Eval243/1(Out1) -> To Workspace243/1
  [in7] -> M245/1(CT2)
  [in8] -> M245/2(F2)
  [in9] -> M245/3(E2)
  [in10] -> M245/4(MR2)
  [in11] -> M245/5(T2)
  [in12] -> M245/6(EB2)
  [in13] -> M245/7(CT3)
  [in14] -> M245/8(F3)
  [in15] -> M245/9(E3)
  [in16] -> M245/10(MR3)
  [in17] -> M245/11(T3)
  [in18] -> M245/12(EB3)
  M245/1(LL2) -> Eval244/1(In2)
  M245/2(LL3) -> Eval244/2(In3)
  Eval244/1(Out1) -> To Workspace244/1
  [in7] -> M246/1(CT2)
  [in8] -> M246/2(F2)
  [in9] -> M246/3(E2)
  [in10] -> M246/4(MR2)
  [in11] -> M246/5(T2)
  [in12] -> M246/6(EB2)
  [in13] -> M246/7(CT3)
  [in14] -> M246/8(F3)
  [in15] -> M246/9(E3)
  [in16] -> M246/10(MR3)
  [in17] -> M246/11(T3)
  [in18] -> M246/12(EB3)
  M246/1(LL2) -> Eval245/1(In2)
  M246/2(LL3) -> Eval245/2(In3)
  Eval245/1(Out1) -> To Workspace245/1
  Inputs/1(CT2) -> dtc_CT2/1
  dtc_CT2/1 -> CPSUT/1(CT2), [in7]
  Inputs/2(F2) -> dtc_F2/1
  dtc_F2/1 -> CPSUT/2(F2), [in8]
  Inputs/3(E2) -> dtc_E2/1
  dtc_E2/1 -> CPSUT/3(E2), [in9]
  Inputs/4(MR2) -> dtc_MR2/1
  dtc_MR2/1 -> CPSUT/4(MR2), [in10]
  Inputs/5(T2) -> dtc_T2/1
  dtc_T2/1 -> CPSUT/5(T2), [in11]
  Inputs/6(EB2) -> dtc_EB2/1
  dtc_EB2/1 -> CPSUT/6(EB2), [in12]
  Inputs/7(CT3) -> dtc_CT3/1
  dtc_CT3/1 -> CPSUT/7(CT3), [in13]
  Inputs/8(F3) -> dtc_F3/1
  dtc_F3/1 -> CPSUT/8(F3), [in14]
  Inputs/9(E3) -> dtc_E3/1
  dtc_E3/1 -> CPSUT/9(E3), [in15]
  Inputs/10(MR3) -> dtc_MR3/1
  dtc_MR3/1 -> CPSUT/10(MR3), [in16]
  Inputs/11(T3) -> dtc_T3/1
  dtc_T3/1 -> CPSUT/11(T3), [in17]
  Inputs/12(EB3) -> dtc_EB3/1
  dtc_EB3/1 -> CPSUT/12(EB3), [in18]
